simulink model "myo_sfun_one_myo_imu_emg"  (R2019a)
(part 7 of 12)

  "IW{2,1}(59,:)'" : Constant  Value=[0.495840889179216037785380422064918093383312225341796875;1.1802197945522425737152616420644335448741912841796875;0.561954816977624727059037468279711902141571044921875;-1.53262922594306960633048220188356935977935791015625;-1.142041866402901728605456810328178107738494873046875;0.444427633542582134484888456427142955362796783447265625;-1.8064715262999488931683345072087831795215606689453125;1.404352830198885460077917741728015244007110595703125]
      mask Display: e = 0.06;c1 = [120 150 230]/255;c2 = ([120 150 230]+0)/383;c3 = ([120 150 230]+128)/383;patch([0 1 1 0],[0 0 1 1],c1);patch([0 1 1 1-e 1-e 0+e],[0 0 1 1-e 0+e 0+e],c2);patch([0 0 1 1-e 0+e 0+e],[0 1 1 1-e 1-e 0+e],c3);plot([0 1 1 0 0],[0 0 1 1 0]);disp('weights');
  "IW{2,1}(590,:)'" : Constant  Value=[1.1365588902599637055601533575099892914295196533203125;-0.7779843835963247133946651956648565828800201416015625;-1.61735271565704774587857173173688352108001708984375;-1.546406279871038957907103394973091781139373779296875;-1.3702407717835847211773625531350262463092803955078125;-0.83551628178603365437737693355302326381206512451171875;0.34674347307820341246298312398721463978290557861328125;1.31964609753725081731090540415607392787933349609375]
      mask Display: e = 0.06;c1 = [120 150 230]/255;c2 = ([120 150 230]+0)/383;c3 = ([120 150 230]+128)/383;patch([0 1 1 0],[0 0 1 1],c1);patch([0 1 1 1-e 1-e 0+e],[0 0 1 1-e 0+e 0+e],c2);patch([0 0 1 1-e 0+e 0+e],[0 1 1 1-e 1-e 0+e],c3);plot([0 1 1 0 0],[0 0 1 1 0]);disp('weights');
  "IW{2,1}(591,:)'" : Constant  Value=[-0.5970468213357691400489102306892164051532745361328125;-0.5252295626150751406413519362104125320911407470703125;0.7731235904409377024393279498326592147350311279296875;1.10843773794026301260373656987212598323822021484375;2.116586324738635394027141956030391156673431396484375;-0.56051950742911482716834825623664073646068572998046875;0.0989810494305454202645933037274517118930816650390625;1.9395521357138549856102827106951735913753509521484375]
      mask Display: e = 0.06;c1 = [120 150 230]/255;c2 = ([120 150 230]+0)/383;c3 = ([120 150 230]+128)/383;patch([0 1 1 0],[0 0 1 1],c1);patch([0 1 1 1-e 1-e 0+e],[0 0 1 1-e 0+e 0+e],c2);patch([0 0 1 1-e 0+e 0+e],[0 1 1 1-e 1-e 0+e],c3);plot([0 1 1 0 0],[0 0 1 1 0]);disp('weights');
  "IW{2,1}(592,:)'" : Constant  Value=[0.56541018625955263843252396327443420886993408203125;-1.92923127145409711857837464776821434497833251953125;-0.11742767155972898274196580814532353542745113372802734375;0.91189640930210702496339081335463561117649078369140625;0.69079553727149856090505863903672434389591217041015625;-1.65512578383373831769631578936241567134857177734375;-1.67777522610076790243738287244923412799835205078125;-0.045770072495004303358978603455398115329444408416748046875]
      mask Display: e = 0.06;c1 = [120 150 230]/255;c2 = ([120 150 230]+0)/383;c3 = ([120 150 230]+128)/383;patch([0 1 1 0],[0 0 1 1],c1);patch([0 1 1 1-e 1-e 0+e],[0 0 1 1-e 0+e 0+e],c2);patch([0 0 1 1-e 0+e 0+e],[0 1 1 1-e 1-e 0+e],c3);plot([0 1 1 0 0],[0 0 1 1 0]);disp('weights');
  "IW{2,1}(593,:)'" : Constant  Value=[1.631995878217446627189701757743023335933685302734375;0.354312519105268231012217938769026659429073333740234375;-0.110400014047913275216927786459564231336116790771484375;1.975595419315174350316510754055343568325042724609375;-0.53976251419960596944491726389969699084758758544921875;-1.4102684742488220681622124175191856920719146728515625;-0.967888206577956378140470405924133956432342529296875;1.0042302158486886565214035726967267692089080810546875]
      mask Display: e = 0.06;c1 = [120 150 230]/255;c2 = ([120 150 230]+0)/383;c3 = ([120 150 230]+128)/383;patch([0 1 1 0],[0 0 1 1],c1);patch([0 1 1 1-e 1-e 0+e],[0 0 1 1-e 0+e 0+e],c2);patch([0 0 1 1-e 0+e 0+e],[0 1 1 1-e 1-e 0+e],c3);plot([0 1 1 0 0],[0 0 1 1 0]);disp('weights');
  "IW{2,1}(594,:)'" : Constant  Value=[1.362855066833854156271854662918485701084136962890625;-1.01753460758354652426760367234237492084503173828125;0.29473268723076551101058839776669628918170928955078125;-0.60966157783774022060896413677255623042583465576171875;-1.3137337831112760877516620894311927258968353271484375;1.764809052114024279234172354335896670818328857421875;1.3718061592596015874079284913023002445697784423828125;0.97264122462135294000518115353770554065704345703125]
      mask Display: e = 0.06;c1 = [120 150 230]/255;c2 = ([120 150 230]+0)/383;c3 = ([120 150 230]+128)/383;patch([0 1 1 0],[0 0 1 1],c1);patch([0 1 1 1-e 1-e 0+e],[0 0 1 1-e 0+e 0+e],c2);patch([0 0 1 1-e 0+e 0+e],[0 1 1 1-e 1-e 0+e],c3);plot([0 1 1 0 0],[0 0 1 1 0]);disp('weights');
  "IW{2,1}(595,:)'" : Constant  Value=[1.7846936263903485642146051759482361376285552978515625;1.17349851398560556248185093863867223262786865234375;1.23537906283144938157647629850544035434722900390625;0.3825987556562269187310221241204999387264251708984375;-1.2332173382475872802643834802438504993915557861328125;0.11657394714668019297665324529589270241558551788330078125;1.813627133167102556399186141788959503173828125;0.0224668411552899037475494736781911342404782772064208984375]
      mask Display: e = 0.06;c1 = [120 150 230]/255;c2 = ([120 150 230]+0)/383;c3 = ([120 150 230]+128)/383;patch([0 1 1 0],[0 0 1 1],c1);patch([0 1 1 1-e 1-e 0+e],[0 0 1 1-e 0+e 0+e],c2);patch([0 0 1 1-e 0+e 0+e],[0 1 1 1-e 1-e 0+e],c3);plot([0 1 1 0 0],[0 0 1 1 0]);disp('weights');
  "IW{2,1}(596,:)'" : Constant  Value=[-2.033022840198186020899129289318807423114776611328125;1.079443546648902074736042777658440172672271728515625;-0.1575933052745503160085860372419119812548160552978515625;-0.547083934928751514092937213717959821224212646484375;1.4229208556832853016516082789166830480098724365234375;-1.5372500566353324291668513978947885334491729736328125;-0.94194300770826944191327356747933663427829742431640625;-0.33000270358517547197862995744799263775348663330078125]
      mask Display: e = 0.06;c1 = [120 150 230]/255;c2 = ([120 150 230]+0)/383;c3 = ([120 150 230]+128)/383;patch([0 1 1 0],[0 0 1 1],c1);patch([0 1 1 1-e 1-e 0+e],[0 0 1 1-e 0+e 0+e],c2);patch([0 0 1 1-e 0+e 0+e],[0 1 1 1-e 1-e 0+e],c3);plot([0 1 1 0 0],[0 0 1 1 0]);disp('weights');
  "IW{2,1}(597,:)'" : Constant  Value=[2.77675076351304550570375795359723269939422607421875;-0.1567492229542953585674780470071709714829921722412109375;0.76572830357359944475348356718313880264759063720703125;-0.13117528257276733771874432932236231863498687744140625;1.034684891448059307350604285602457821369171142578125;0.210211678674975088743082096698344685137271881103515625;-0.987697962369239679247812091489322483539581298828125;0.741366082034913720377744539291597902774810791015625]
      mask Display: e = 0.06;c1 = [120 150 230]/255;c2 = ([120 150 230]+0)/383;c3 = ([120 150 230]+128)/383;patch([0 1 1 0],[0 0 1 1],c1);patch([0 1 1 1-e 1-e 0+e],[0 0 1 1-e 0+e 0+e],c2);patch([0 0 1 1-e 0+e 0+e],[0 1 1 1-e 1-e 0+e],c3);plot([0 1 1 0 0],[0 0 1 1 0]);disp('weights');
  "IW{2,1}(598,:)'" : Constant  Value=[-1.4404722918007439869114705288666300475597381591796875;1.4952177887590389904204357662820257246494293212890625;0.7882227735106985822000069674686528742313385009765625;1.250002842826308135926183240371756255626678466796875;-0.240822773039876258938107866924838162958621978759765625;-1.3647491667626006073277267205412499606609344482421875;-1.4597226525156685728035199645091779530048370361328125;0.7848545039343071128001838587806560099124908447265625]
      mask Display: e = 0.06;c1 = [120 150 230]/255;c2 = ([120 150 230]+0)/383;c3 = ([120 150 230]+128)/383;patch([0 1 1 0],[0 0 1 1],c1);patch([0 1 1 1-e 1-e 0+e],[0 0 1 1-e 0+e 0+e],c2);patch([0 0 1 1-e 0+e 0+e],[0 1 1 1-e 1-e 0+e],c3);plot([0 1 1 0 0],[0 0 1 1 0]);disp('weights');
  "IW{2,1}(599,:)'" : Constant  Value=[1.3324967037313222295580317222629673779010772705078125;1.9427219282712944181668035525945015251636505126953125;-0.246444365406416066033301603965810500085353851318359375;1.03972745733009386270850882283411920070648193359375;0.94374530422070801449763166601769626140594482421875;-1.5873018147496045227029526358819566667079925537109375;0.4525167778451917310889029977261088788509368896484375;-0.8947395514296709873036661520018242299556732177734375]
      mask Display: e = 0.06;c1 = [120 150 230]/255;c2 = ([120 150 230]+0)/383;c3 = ([120 150 230]+128)/383;patch([0 1 1 0],[0 0 1 1],c1);patch([0 1 1 1-e 1-e 0+e],[0 0 1 1-e 0+e 0+e],c2);patch([0 0 1 1-e 0+e 0+e],[0 1 1 1-e 1-e 0+e],c3);plot([0 1 1 0 0],[0 0 1 1 0]);disp('weights');
  "IW{2,1}(6,:)'" : Constant  Value=[1.3989645708381897026839624231797643005847930908203125;0.878871965177622005427338081062771379947662353515625;1.4478398212565826153053194502717815339565277099609375;0.386861724085491631708322302074520848691463470458984375;-1.4881625315723978619786294075311161577701568603515625;1.25220042774751139091904406086541712284088134765625;-1.41799544675611599586773081682622432708740234375;-0.450735541140858231301535852253437042236328125]
      mask Display: e = 0.06;c1 = [120 150 230]/255;c2 = ([120 150 230]+0)/383;c3 = ([120 150 230]+128)/383;patch([0 1 1 0],[0 0 1 1],c1);patch([0 1 1 1-e 1-e 0+e],[0 0 1 1-e 0+e 0+e],c2);patch([0 0 1 1-e 0+e 0+e],[0 1 1 1-e 1-e 0+e],c3);plot([0 1 1 0 0],[0 0 1 1 0]);disp('weights');
  "IW{2,1}(60,:)'" : Constant  Value=[-1.56723963251996156742507082526572048664093017578125;-1.8273391712930813213233705027960240840911865234375;0.062222286282019624581440808697152533568441867828369140625;0.489904984279520616663461396456114016473293304443359375;0.263246879203439199113034874244476668536663055419921875;-1.783690226821929680767198078683577477931976318359375;-0.3950211766085482967270081644528545439243316650390625;-1.305120998374337037972736652591265738010406494140625]
      mask Display: e = 0.06;c1 = [120 150 230]/255;c2 = ([120 150 230]+0)/383;c3 = ([120 150 230]+128)/383;patch([0 1 1 0],[0 0 1 1],c1);patch([0 1 1 1-e 1-e 0+e],[0 0 1 1-e 0+e 0+e],c2);patch([0 0 1 1-e 0+e 0+e],[0 1 1 1-e 1-e 0+e],c3);plot([0 1 1 0 0],[0 0 1 1 0]);disp('weights');
  "IW{2,1}(600,:)'" : Constant  Value=[0.1399013578316503358944800083918380551040172576904296875;0.994745433658990041436709361732937395572662353515625;0.07987948964757167480410515736366505734622478485107421875;-1.1014921740343570633058334351517260074615478515625;0.90693688484948487005254946780041791498661041259765625;-2.023313920340508165196524714701808989048004150390625;0.2991665154529716819098439373192377388477325439453125;1.9577441671871154138528936528018675744533538818359375]
      mask Display: e = 0.06;c1 = [120 150 230]/255;c2 = ([120 150 230]+0)/383;c3 = ([120 150 230]+128)/383;patch([0 1 1 0],[0 0 1 1],c1);patch([0 1 1 1-e 1-e 0+e],[0 0 1 1-e 0+e 0+e],c2);patch([0 0 1 1-e 0+e 0+e],[0 1 1 1-e 1-e 0+e],c3);plot([0 1 1 0 0],[0 0 1 1 0]);disp('weights');
  "IW{2,1}(601,:)'" : Constant  Value=[-1.0462262509493889250933307266677729785442352294921875;-1.363451040177134476749642999493516981601715087890625;-1.3802141630787783110889677118393592536449432373046875;-1.4657412561269500539395949090248905122280120849609375;1.27038054359856733555034224991686642169952392578125;-0.59673781341977327752346127454075030982494354248046875;1.4209709404646198027677428399329073727130889892578125;0.186387720666462197716128912361455149948596954345703125]
      mask Display: e = 0.06;c1 = [120 150 230]/255;c2 = ([120 150 230]+0)/383;c3 = ([120 150 230]+128)/383;patch([0 1 1 0],[0 0 1 1],c1);patch([0 1 1 1-e 1-e 0+e],[0 0 1 1-e 0+e 0+e],c2);patch([0 0 1 1-e 0+e 0+e],[0 1 1 1-e 1-e 0+e],c3);plot([0 1 1 0 0],[0 0 1 1 0]);disp('weights');
  "IW{2,1}(602,:)'" : Constant  Value=[1.0676591676437723332782070428947918117046356201171875;-1.1515456246222381953003832677495665848255157470703125;1.199234109027186523377395133138634264469146728515625;1.1004753429431255451476090456708334386348724365234375;0.348101446973952344254854551763855852186679840087890625;1.257095724948527060149672252009622752666473388671875;1.536305124972318747467170396703295409679412841796875;1.3476924591500065719884560166974551975727081298828125]
      mask Display: e = 0.06;c1 = [120 150 230]/255;c2 = ([120 150 230]+0)/383;c3 = ([120 150 230]+128)/383;patch([0 1 1 0],[0 0 1 1],c1);patch([0 1 1 1-e 1-e 0+e],[0 0 1 1-e 0+e 0+e],c2);patch([0 0 1 1-e 0+e 0+e],[0 1 1 1-e 1-e 0+e],c3);plot([0 1 1 0 0],[0 0 1 1 0]);disp('weights');
  "IW{2,1}(603,:)'" : Constant  Value=[-0.8102015609143695673566298864898271858692169189453125;0.9788842783427773586168996189371682703495025634765625;-0.546574779209751948627626916277222335338592529296875;-1.380296283345530117259158942033536732196807861328125;-1.3637937080773421261170597063028253614902496337890625;1.5946411678625553864918629187741316854953765869140625;0.94363969580705742146164993755519390106201171875;-1.43620112704588986929366001277230679988861083984375]
      mask Display: e = 0.06;c1 = [120 150 230]/255;c2 = ([120 150 230]+0)/383;c3 = ([120 150 230]+128)/383;patch([0 1 1 0],[0 0 1 1],c1);patch([0 1 1 1-e 1-e 0+e],[0 0 1 1-e 0+e 0+e],c2);patch([0 0 1 1-e 0+e 0+e],[0 1 1 1-e 1-e 0+e],c3);plot([0 1 1 0 0],[0 0 1 1 0]);disp('weights');
  "IW{2,1}(604,:)'" : Constant  Value=[0.406274079118545572431031587257166393101215362548828125;-1.0380674950344452867057043476961553096771240234375;1.3401458758174744634317221425590105354785919189453125;-0.44440858715460251904261212985147722065448760986328125;0.97805948319445568106544897091225720942020416259765625;-1.065572892148696215741665582754649221897125244140625;1.7562937018632605035151073025190271437168121337890625;-1.6116834669183486283827733132056891918182373046875]
      mask Display: e = 0.06;c1 = [120 150 230]/255;c2 = ([120 150 230]+0)/383;c3 = ([120 150 230]+128)/383;patch([0 1 1 0],[0 0 1 1],c1);patch([0 1 1 1-e 1-e 0+e],[0 0 1 1-e 0+e 0+e],c2);patch([0 0 1 1-e 0+e 0+e],[0 1 1 1-e 1-e 0+e],c3);plot([0 1 1 0 0],[0 0 1 1 0]);disp('weights');
  "IW{2,1}(605,:)'" : Constant  Value=[0.744501259166927109589551037061028182506561279296875;-1.160653386032304279495974697056226432323455810546875;1.663776115535684052559872725396417081356048583984375;0.08145048492487029501152306920630508102476596832275390625;1.5551761046942977895213289230014197528362274169921875;1.6110581647783417391650573335937224328517913818359375;-0.77332975038642615128736679253051988780498504638671875;-0.86635308081110107281119780964218080043792724609375]
      mask Display: e = 0.06;c1 = [120 150 230]/255;c2 = ([120 150 230]+0)/383;c3 = ([120 150 230]+128)/383;patch([0 1 1 0],[0 0 1 1],c1);patch([0 1 1 1-e 1-e 0+e],[0 0 1 1-e 0+e 0+e],c2);patch([0 0 1 1-e 0+e 0+e],[0 1 1 1-e 1-e 0+e],c3);plot([0 1 1 0 0],[0 0 1 1 0]);disp('weights');
  "IW{2,1}(606,:)'" : Constant  Value=[-2.00759017283681817644946931977756321430206298828125;1.4790292348892355445144630721188150346279144287109375;0.9381068897441531273528880774392746388912200927734375;-1.0279233837163934683900379241094924509525299072265625;1.530338655101361577948182457475923001766204833984375;0.70558561888594562017118505536927841603755950927734375;-0.389949820912730060751272276320378296077251434326171875;-0.30903615573059750598616801653406582772731781005859375]
      mask Display: e = 0.06;c1 = [120 150 230]/255;c2 = ([120 150 230]+0)/383;c3 = ([120 150 230]+128)/383;patch([0 1 1 0],[0 0 1 1],c1);patch([0 1 1 1-e 1-e 0+e],[0 0 1 1-e 0+e 0+e],c2);patch([0 0 1 1-e 0+e 0+e],[0 1 1 1-e 1-e 0+e],c3);plot([0 1 1 0 0],[0 0 1 1 0]);disp('weights');
  "IW{2,1}(607,:)'" : Constant  Value=[-1.0176822149305377873673705835244618356227874755859375;-0.88067083235813570230021696261246688663959503173828125;-1.2233134249827359862905495901941321790218353271484375;1.6120984193939709161469409082201309502124786376953125;-0.01641788180701951593842835563918924890458583831787109375;1.842094851055680493345789727754890918731689453125;0.387559764525972905158113235302153043448925018310546875;-1.28754911299864627238775938167236745357513427734375]
      mask Display: e = 0.06;c1 = [120 150 230]/255;c2 = ([120 150 230]+0)/383;c3 = ([120 150 230]+128)/383;patch([0 1 1 0],[0 0 1 1],c1);patch([0 1 1 1-e 1-e 0+e],[0 0 1 1-e 0+e 0+e],c2);patch([0 0 1 1-e 0+e 0+e],[0 1 1 1-e 1-e 0+e],c3);plot([0 1 1 0 0],[0 0 1 1 0]);disp('weights');
  "IW{2,1}(608,:)'" : Constant  Value=[0.06756783426557622096453314952668733894824981689453125;-0.97985811135812161953850818463251926004886627197265625;1.9165656766479255423973881988786160945892333984375;0.97999553847674636397613312510657124221324920654296875;1.0965168003811542885017615844844840466976165771484375;0.91483034898736093065707564164767973124980926513671875;0.416384344635610970097872041151276789605617523193359375;-1.8438560716209162482215333511703647673130035400390625]
      mask Display: e = 0.06;c1 = [120 150 230]/255;c2 = ([120 150 230]+0)/383;c3 = ([120 150 230]+128)/383;patch([0 1 1 0],[0 0 1 1],c1);patch([0 1 1 1-e 1-e 0+e],[0 0 1 1-e 0+e 0+e],c2);patch([0 0 1 1-e 0+e 0+e],[0 1 1 1-e 1-e 0+e],c3);plot([0 1 1 0 0],[0 0 1 1 0]);disp('weights');
  "IW{2,1}(609,:)'" : Constant  Value=[0.90824883915620002738933180808089673519134521484375;1.5432188808015123715478011945378966629505157470703125;-0.484591429101132231682669271322083659470081329345703125;-0.75644137307587389074114980758167803287506103515625;-1.4204857677377356051096057854010723531246185302734375;1.5424089274776846547609920889954082667827606201171875;-1.3677706917546246234707041367073543369770050048828125;0.67875477880856471823989295444334857165813446044921875]
      mask Display: e = 0.06;c1 = [120 150 230]/255;c2 = ([120 150 230]+0)/383;c3 = ([120 150 230]+128)/383;patch([0 1 1 0],[0 0 1 1],c1);patch([0 1 1 1-e 1-e 0+e],[0 0 1 1-e 0+e 0+e],c2);patch([0 0 1 1-e 0+e 0+e],[0 1 1 1-e 1-e 0+e],c3);plot([0 1 1 0 0],[0 0 1 1 0]);disp('weights');
  "IW{2,1}(61,:)'" : Constant  Value=[-0.583346229666195537078010602272115647792816162109375;0.652606918201581009952860767953097820281982421875;1.54396791785674469821287857485003769397735595703125;-0.8547845495893435785461633713566698133945465087890625;1.440314162861167091023162356577813625335693359375;0.48672290195644507537764411608804948627948760986328125;-1.430158866254590321887008030898869037628173828125;1.66829878736194192612174447276629507541656494140625]
      mask Display: e = 0.06;c1 = [120 150 230]/255;c2 = ([120 150 230]+0)/383;c3 = ([120 150 230]+128)/383;patch([0 1 1 0],[0 0 1 1],c1);patch([0 1 1 1-e 1-e 0+e],[0 0 1 1-e 0+e 0+e],c2);patch([0 0 1 1-e 0+e 0+e],[0 1 1 1-e 1-e 0+e],c3);plot([0 1 1 0 0],[0 0 1 1 0]);disp('weights');
  "IW{2,1}(610,:)'" : Constant  Value=[1.0695065922145297054868251507286913692951202392578125;-0.5602414711219931842123287424328736960887908935546875;1.564508360252296004233585335896350443363189697265625;0.443578046982452567359445083639002405107021331787109375;1.8320578553493607198987547235446982085704803466796875;0.2373867145462984218351465415253187529742717742919921875;-1.4201256732646430069877396817901171743869781494140625;-1.230718785601741416257937089540064334869384765625]
      mask Display: e = 0.06;c1 = [120 150 230]/255;c2 = ([120 150 230]+0)/383;c3 = ([120 150 230]+128)/383;patch([0 1 1 0],[0 0 1 1],c1);patch([0 1 1 1-e 1-e 0+e],[0 0 1 1-e 0+e 0+e],c2);patch([0 0 1 1-e 0+e 0+e],[0 1 1 1-e 1-e 0+e],c3);plot([0 1 1 0 0],[0 0 1 1 0]);disp('weights');
  "IW{2,1}(611,:)'" : Constant  Value=[-0.56186312548356831531037869353895075619220733642578125;1.9518020246530098926740492970566265285015106201171875;-0.94334391080466650780778081752941943705081939697265625;-1.9538154513649264032437713467516005039215087890625;0.109136425671035930395902369127725251019001007080078125;-0.528305999598769115976892862818203866481781005859375;0.8902645159678039821216088967048563063144683837890625;1.022948550793317590290598673163913190364837646484375]
      mask Display: e = 0.06;c1 = [120 150 230]/255;c2 = ([120 150 230]+0)/383;c3 = ([120 150 230]+128)/383;patch([0 1 1 0],[0 0 1 1],c1);patch([0 1 1 1-e 1-e 0+e],[0 0 1 1-e 0+e 0+e],c2);patch([0 0 1 1-e 0+e 0+e],[0 1 1 1-e 1-e 0+e],c3);plot([0 1 1 0 0],[0 0 1 1 0]);disp('weights');
  "IW{2,1}(612,:)'" : Constant  Value=[-1.19478104240437144056841134442947804927825927734375;2.162698980018332495234290036023594439029693603515625;-0.693116982716233120953575053135864436626434326171875;1.2670612929229212451076591605669818818569183349609375;1.154640366877071944173849260550923645496368408203125;-0.618604838251085364930759169510565698146820068359375;0.318475683817145138743143206738750450313091278076171875;-0.99402698682691192910709787611267529428005218505859375]
      mask Display: e = 0.06;c1 = [120 150 230]/255;c2 = ([120 150 230]+0)/383;c3 = ([120 150 230]+128)/383;patch([0 1 1 0],[0 0 1 1],c1);patch([0 1 1 1-e 1-e 0+e],[0 0 1 1-e 0+e 0+e],c2);patch([0 0 1 1-e 0+e 0+e],[0 1 1 1-e 1-e 0+e],c3);plot([0 1 1 0 0],[0 0 1 1 0]);disp('weights');
  "IW{2,1}(613,:)'" : Constant  Value=[1.5390431098582713076439176802523434162139892578125;0.311842151138437662094560209880000911653041839599609375;-0.432826553257930901619232599841780029237270355224609375;-1.135667286790710051036512595601379871368408203125;-1.2510952563992765451672539711580611765384674072265625;-1.099051054945733074674762974609620869159698486328125;-1.314184632408988750995604277704842388629913330078125;-1.5719194667600806525342704844661056995391845703125]
      mask Display: e = 0.06;c1 = [120 150 230]/255;c2 = ([120 150 230]+0)/383;c3 = ([120 150 230]+128)/383;patch([0 1 1 0],[0 0 1 1],c1);patch([0 1 1 1-e 1-e 0+e],[0 0 1 1-e 0+e 0+e],c2);patch([0 0 1 1-e 0+e 0+e],[0 1 1 1-e 1-e 0+e],c3);plot([0 1 1 0 0],[0 0 1 1 0]);disp('weights');
  "IW{2,1}(614,:)'" : Constant  Value=[0.415642840330518958946726115755154751241207122802734375;1.47348021001815165931247975095175206661224365234375;0.5290336561264969983398032127297483384609222412109375;-1.3355131601420442422067935694940388202667236328125;1.91821924338969385104292086907662451267242431640625;0.598986782930229555432788401958532631397247314453125;-1.395334022050206623788426441024057567119598388671875;-0.83432116509932086056977595944772474467754364013671875]
      mask Display: e = 0.06;c1 = [120 150 230]/255;c2 = ([120 150 230]+0)/383;c3 = ([120 150 230]+128)/383;patch([0 1 1 0],[0 0 1 1],c1);patch([0 1 1 1-e 1-e 0+e],[0 0 1 1-e 0+e 0+e],c2);patch([0 0 1 1-e 0+e 0+e],[0 1 1 1-e 1-e 0+e],c3);plot([0 1 1 0 0],[0 0 1 1 0]);disp('weights');
  "IW{2,1}(615,:)'" : Constant  Value=[-0.9243394765822106062813645621645264327526092529296875;2.523292336225384957515416317619383335113525390625;-0.497732778806864839538093292503617703914642333984375;1.3000054053377587681694649290875531733036041259765625;0.8499300349543557064890819674474187195301055908203125;0.86402793265875355022131998339318670332431793212890625;-0.57755068516618124352390850617666728794574737548828125;0.1895537067373020134741778974785120226442813873291015625]
      mask Display: e = 0.06;c1 = [120 150 230]/255;c2 = ([120 150 230]+0)/383;c3 = ([120 150 230]+128)/383;patch([0 1 1 0],[0 0 1 1],c1);patch([0 1 1 1-e 1-e 0+e],[0 0 1 1-e 0+e 0+e],c2);patch([0 0 1 1-e 0+e 0+e],[0 1 1 1-e 1-e 0+e],c3);plot([0 1 1 0 0],[0 0 1 1 0]);disp('weights');
  "IW{2,1}(616,:)'" : Constant  Value=[-1.7980650129034174700137782565434463322162628173828125;-0.52787175708551858921424582149484194815158843994140625;0.3999021950203929254286094874260015785694122314453125;1.2856492697510863987275797626352868974208831787109375;-0.8074119078345536326679621197399683296680450439453125;1.0282666253705297076947999812546186149120330810546875;1.5670907494630854639439121456234715878963470458984375;1.2173301229011121993295319043681956827640533447265625]
      mask Display: e = 0.06;c1 = [120 150 230]/255;c2 = ([120 150 230]+0)/383;c3 = ([120 150 230]+128)/383;patch([0 1 1 0],[0 0 1 1],c1);patch([0 1 1 1-e 1-e 0+e],[0 0 1 1-e 0+e 0+e],c2);patch([0 0 1 1-e 0+e 0+e],[0 1 1 1-e 1-e 0+e],c3);plot([0 1 1 0 0],[0 0 1 1 0]);disp('weights');
  "IW{2,1}(617,:)'" : Constant  Value=[0.8233944981282481645479265353060327470302581787109375;2.07864078264244600546817309805192053318023681640625;0.97238679166842933998538001105771400034427642822265625;-0.7199181388481150634106597863137722015380859375;0.421549209390107371131506397432531230151653289794921875;-1.1523597959586282524213629585574381053447723388671875;-0.425262518672025635613209715302218683063983917236328125;-1.6941255159399364327299508659052662551403045654296875]
      mask Display: e = 0.06;c1 = [120 150 230]/255;c2 = ([120 150 230]+0)/383;c3 = ([120 150 230]+128)/383;patch([0 1 1 0],[0 0 1 1],c1);patch([0 1 1 1-e 1-e 0+e],[0 0 1 1-e 0+e 0+e],c2);patch([0 0 1 1-e 0+e 0+e],[0 1 1 1-e 1-e 0+e],c3);plot([0 1 1 0 0],[0 0 1 1 0]);disp('weights');
  "IW{2,1}(618,:)'" : Constant  Value=[-1.3845112013980223064635310947778634727001190185546875;1.2581019145671932246699498136877082288265228271484375;0.385219614654531194997133525248500518500804901123046875;-0.378698122941593329215947960619814693927764892578125;1.6636808845950714630390621096012182533740997314453125;-1.326437238051724865073310866137035191059112548828125;-0.4094163915923871854829485528171062469482421875;1.599983886636860308527730012428946793079376220703125]
      mask Display: e = 0.06;c1 = [120 150 230]/255;c2 = ([120 150 230]+0)/383;c3 = ([120 150 230]+128)/383;patch([0 1 1 0],[0 0 1 1],c1);patch([0 1 1 1-e 1-e 0+e],[0 0 1 1-e 0+e 0+e],c2);patch([0 0 1 1-e 0+e 0+e],[0 1 1 1-e 1-e 0+e],c3);plot([0 1 1 0 0],[0 0 1 1 0]);disp('weights');
  "IW{2,1}(619,:)'" : Constant  Value=[1.6832996710298167020170012619928456842899322509765625;0.449539198982113585856268400675617158412933349609375;0.8307320998601823713869407583842985332012176513671875;-0.6832544444925467974627508738194592297077178955078125;-2.2669423406538786736064139404334127902984619140625;-0.21058789806763034135883572162128984928131103515625;-0.93104019495121892457945023124921135604381561279296875;-0.94874025383826599000514079307322390377521514892578125]
      mask Display: e = 0.06;c1 = [120 150 230]/255;c2 = ([120 150 230]+0)/383;c3 = ([120 150 230]+128)/383;patch([0 1 1 0],[0 0 1 1],c1);patch([0 1 1 1-e 1-e 0+e],[0 0 1 1-e 0+e 0+e],c2);patch([0 0 1 1-e 0+e 0+e],[0 1 1 1-e 1-e 0+e],c3);plot([0 1 1 0 0],[0 0 1 1 0]);disp('weights');
  "IW{2,1}(62,:)'" : Constant  Value=[-0.80784071268572432700239005498588085174560546875;-0.86454159290918097813261056217015720903873443603515625;-1.02798280810631492698803413077257573604583740234375;-0.843159200916097528732962018693797290325164794921875;1.9764345113544423693241469663917087018489837646484375;-1.0226218063283021297849018083070404827594757080078125;1.3440794621918434881280290937866084277629852294921875;-1.0325956562448708186963131083757616579532623291015625]
      mask Display: e = 0.06;c1 = [120 150 230]/255;c2 = ([120 150 230]+0)/383;c3 = ([120 150 230]+128)/383;patch([0 1 1 0],[0 0 1 1],c1);patch([0 1 1 1-e 1-e 0+e],[0 0 1 1-e 0+e 0+e],c2);patch([0 0 1 1-e 0+e 0+e],[0 1 1 1-e 1-e 0+e],c3);plot([0 1 1 0 0],[0 0 1 1 0]);disp('weights');
  "IW{2,1}(620,:)'" : Constant  Value=[1.334947324367666166011758832610212266445159912109375;-1.3273493586359659257567500389995984733104705810546875;-0.1321542017070956587243557578403851948678493499755859375;-1.294590725841910927584876844775862991809844970703125;1.4144908241846343432968069464550353586673736572265625;-0.4990548052459355954368902530404739081859588623046875;-1.14994285385152839040756589383818209171295166015625;-1.4414002009392941072718485884252004325389862060546875]
      mask Display: e = 0.06;c1 = [120 150 230]/255;c2 = ([120 150 230]+0)/383;c3 = ([120 150 230]+128)/383;patch([0 1 1 0],[0 0 1 1],c1);patch([0 1 1 1-e 1-e 0+e],[0 0 1 1-e 0+e 0+e],c2);patch([0 0 1 1-e 0+e 0+e],[0 1 1 1-e 1-e 0+e],c3);plot([0 1 1 0 0],[0 0 1 1 0]);disp('weights');
  "IW{2,1}(621,:)'" : Constant  Value=[-0.1155194033765267469515691800552303902804851531982421875;-0.344314053861413338353258950519375503063201904296875;-0.18025558100015171003605018995585851371288299560546875;1.66092833072870948996069273562170565128326416015625;0.5727993422400086132029173313640058040618896484375;1.389429199332991249349333884310908615589141845703125;0.5034936486076386774612956287455745041370391845703125;-2.326123140285625279233272522105835378170013427734375]
      mask Display: e = 0.06;c1 = [120 150 230]/255;c2 = ([120 150 230]+0)/383;c3 = ([120 150 230]+128)/383;patch([0 1 1 0],[0 0 1 1],c1);patch([0 1 1 1-e 1-e 0+e],[0 0 1 1-e 0+e 0+e],c2);patch([0 0 1 1-e 0+e 0+e],[0 1 1 1-e 1-e 0+e],c3);plot([0 1 1 0 0],[0 0 1 1 0]);disp('weights');
  "IW{2,1}(622,:)'" : Constant  Value=[-0.327523627563958752428874277029535733163356781005859375;-1.3950088720842390710430436229216866195201873779296875;-0.07732020025750445391121701277370448224246501922607421875;-1.1070020699473712699756333677214570343494415283203125;1.3609328905626727479472037884988822042942047119140625;1.5808360841818320796647867609863169491291046142578125;1.00853180773224249122677065315656363964080810546875;1.49164411309901101532204847899265587329864501953125]
      mask Display: e = 0.06;c1 = [120 150 230]/255;c2 = ([120 150 230]+0)/383;c3 = ([120 150 230]+128)/383;patch([0 1 1 0],[0 0 1 1],c1);patch([0 1 1 1-e 1-e 0+e],[0 0 1 1-e 0+e 0+e],c2);patch([0 0 1 1-e 0+e 0+e],[0 1 1 1-e 1-e 0+e],c3);plot([0 1 1 0 0],[0 0 1 1 0]);disp('weights');
  "IW{2,1}(623,:)'" : Constant  Value=[0.50926268929817919417502025680732913315296173095703125;1.02354553421339034002812695689499378204345703125;0.4587054237810974655076279304921627044677734375;-1.2664756748000687291977328641223721206188201904296875;-1.0326915158366702929271241373498924076557159423828125;0.404808695052300715477855419521802105009555816650390625;1.7725295585873281911659660181612707674503326416015625;-1.9056231855257212970400360063649713993072509765625]
      mask Display: e = 0.06;c1 = [120 150 230]/255;c2 = ([120 150 230]+0)/383;c3 = ([120 150 230]+128)/383;patch([0 1 1 0],[0 0 1 1],c1);patch([0 1 1 1-e 1-e 0+e],[0 0 1 1-e 0+e 0+e],c2);patch([0 0 1 1-e 0+e 0+e],[0 1 1 1-e 1-e 0+e],c3);plot([0 1 1 0 0],[0 0 1 1 0]);disp('weights');
  "IW{2,1}(624,:)'" : Constant  Value=[-0.426022704578880306858224003008217550814151763916015625;1.974465496821880439171081889071501791477203369140625;0.34657118674579923123246771865524351596832275390625;0.97614887195124910856947053616750054061412811279296875;-1.4175229737882946157156993649550713598728179931640625;-1.33353469225431897626776844845153391361236572265625;0.51150649856705754370267413833062164485454559326171875;-1.3644009071495613039104455310734920203685760498046875]
      mask Display: e = 0.06;c1 = [120 150 230]/255;c2 = ([120 150 230]+0)/383;c3 = ([120 150 230]+128)/383;patch([0 1 1 0],[0 0 1 1],c1);patch([0 1 1 1-e 1-e 0+e],[0 0 1 1-e 0+e 0+e],c2);patch([0 0 1 1-e 0+e 0+e],[0 1 1 1-e 1-e 0+e],c3);plot([0 1 1 0 0],[0 0 1 1 0]);disp('weights');
  "IW{2,1}(625,:)'" : Constant  Value=[1.0892807111617666127045822577201761305332183837890625;1.962879653505605670460454348358325660228729248046875;-0.4366435090927993645237847886164672672748565673828125;-1.499077208754342915852930673281662166118621826171875;-1.062067905261328437660495183081366121768951416015625;0.64284583767381631158599475384107790887355804443359375;1.320911793095183472956932746456004679203033447265625;-0.540715402800169275820962866418994963169097900390625]
      mask Display: e = 0.06;c1 = [120 150 230]/255;c2 = ([120 150 230]+0)/383;c3 = ([120 150 230]+128)/383;patch([0 1 1 0],[0 0 1 1],c1);patch([0 1 1 1-e 1-e 0+e],[0 0 1 1-e 0+e 0+e],c2);patch([0 0 1 1-e 0+e 0+e],[0 1 1 1-e 1-e 0+e],c3);plot([0 1 1 0 0],[0 0 1 1 0]);disp('weights');
  "IW{2,1}(626,:)'" : Constant  Value=[-0.0934478463088293798133321388377225957810878753662109375;0.364146124661070602623880176906823180615901947021484375;1.54354569628061089048287612968124449253082275390625;1.1389569591664339132108807461918331682682037353515625;1.551203771758578486839041943312622606754302978515625;-1.5252177846193613053316084915422834455966949462890625;1.4405943699840950689150531616178341209888458251953125;0.70619852150084183595168951796949841082096099853515625]
      mask Display: e = 0.06;c1 = [120 150 230]/255;c2 = ([120 150 230]+0)/383;c3 = ([120 150 230]+128)/383;patch([0 1 1 0],[0 0 1 1],c1);patch([0 1 1 1-e 1-e 0+e],[0 0 1 1-e 0+e 0+e],c2);patch([0 0 1 1-e 0+e 0+e],[0 1 1 1-e 1-e 0+e],c3);plot([0 1 1 0 0],[0 0 1 1 0]);disp('weights');
  "IW{2,1}(627,:)'" : Constant  Value=[0.09219685402307654931153280131184146739542484283447265625;0.07017065301976861679822405903905746527016162872314453125;1.52843238753498145143794317846186459064483642578125;0.965812028758090246327583372476510703563690185546875;2.112261949203092736837561460561119019985198974609375;0.07524462289875240295078384633598034270107746124267578125;1.751589707715766497386766786803491413593292236328125;0.43357744552148413941239368796232156455516815185546875]
      mask Display: e = 0.06;c1 = [120 150 230]/255;c2 = ([120 150 230]+0)/383;c3 = ([120 150 230]+128)/383;patch([0 1 1 0],[0 0 1 1],c1);patch([0 1 1 1-e 1-e 0+e],[0 0 1 1-e 0+e 0+e],c2);patch([0 0 1 1-e 0+e 0+e],[0 1 1 1-e 1-e 0+e],c3);plot([0 1 1 0 0],[0 0 1 1 0]);disp('weights');
  "IW{2,1}(628,:)'" : Constant  Value=[1.6577552297238258294242996271350421011447906494140625;0.51268986432709573453081475236103869974613189697265625;-1.4036568104439470783262322584050707519054412841796875;0.9921396182445401112914851182722486555576324462890625;-1.53525969285640417894001075183041393756866455078125;1.2058938538982564292467714039958082139492034912109375;0.051529486221002528123502628432106575928628444671630859375;1.091902940613427741567420525825582444667816162109375]
      mask Display: e = 0.06;c1 = [120 150 230]/255;c2 = ([120 150 230]+0)/383;c3 = ([120 150 230]+128)/383;patch([0 1 1 0],[0 0 1 1],c1);patch([0 1 1 1-e 1-e 0+e],[0 0 1 1-e 0+e 0+e],c2);patch([0 0 1 1-e 0+e 0+e],[0 1 1 1-e 1-e 0+e],c3);plot([0 1 1 0 0],[0 0 1 1 0]);disp('weights');
  "IW{2,1}(629,:)'" : Constant  Value=[1.2589993845590898846609206884750165045261383056640625;1.4979357158170494290772012391244061291217803955078125;-0.90621099390727610778384359946358017623424530029296875;0.97946455928432885063017465654411353170871734619140625;-1.0229675550841654807499025992001406848430633544921875;-1.548306923334317186657926868065260350704193115234375;1.281460062898937213304861870710738003253936767578125;-0.58596677840527833236450305776088498532772064208984375]
      mask Display: e = 0.06;c1 = [120 150 230]/255;c2 = ([120 150 230]+0)/383;c3 = ([120 150 230]+128)/383;patch([0 1 1 0],[0 0 1 1],c1);patch([0 1 1 1-e 1-e 0+e],[0 0 1 1-e 0+e 0+e],c2);patch([0 0 1 1-e 0+e 0+e],[0 1 1 1-e 1-e 0+e],c3);plot([0 1 1 0 0],[0 0 1 1 0]);disp('weights');
  "IW{2,1}(63,:)'" : Constant  Value=[-0.7144457458977411246081601348123513162136077880859375;-0.007298700002133218060762498424764999072067439556121826171875;1.44780006772763325528785571805201470851898193359375;-1.788137173619348541109275174676440656185150146484375;-1.58123753756977425410923387971706688404083251953125;1.55199278995771106082202095421962440013885498046875;-0.5036095123205377444008945531095378100872039794921875;0.09057178325152830111743895713516394607722759246826171875]
      mask Display: e = 0.06;c1 = [120 150 230]/255;c2 = ([120 150 230]+0)/383;c3 = ([120 150 230]+128)/383;patch([0 1 1 0],[0 0 1 1],c1);patch([0 1 1 1-e 1-e 0+e],[0 0 1 1-e 0+e 0+e],c2);patch([0 0 1 1-e 0+e 0+e],[0 1 1 1-e 1-e 0+e],c3);plot([0 1 1 0 0],[0 0 1 1 0]);disp('weights');
  "IW{2,1}(630,:)'" : Constant  Value=[0.0982183466709679320327808227375498972833156585693359375;-0.1268629177400806273823263836675323545932769775390625;-0.300995077456217341449473678949289023876190185546875;2.173761256513340622831265136483125388622283935546875;-1.5145394274333738859894538109074346721172332763671875;1.60123112841297920994065862032584846019744873046875;-0.140390045149285602743560730232275091111660003662109375;1.1047487791690600023031265664030797779560089111328125]
      mask Display: e = 0.06;c1 = [120 150 230]/255;c2 = ([120 150 230]+0)/383;c3 = ([120 150 230]+128)/383;patch([0 1 1 0],[0 0 1 1],c1);patch([0 1 1 1-e 1-e 0+e],[0 0 1 1-e 0+e 0+e],c2);patch([0 0 1 1-e 0+e 0+e],[0 1 1 1-e 1-e 0+e],c3);plot([0 1 1 0 0],[0 0 1 1 0]);disp('weights');
  "IW{2,1}(631,:)'" : Constant  Value=[1.3164862241914558893540743156336247920989990234375;-0.468865499463230361865129225407144986093044281005859375;-1.12740594557454887336689353105612099170684814453125;0.61935334953164922211499288096092641353607177734375;-1.809596865877384885834544547833502292633056640625;-0.86133225167429461333057361116516403853893280029296875;-0.50304123527349775546468890752294100821018218994140625;-1.7703580003685785992928458654205314815044403076171875]
      mask Display: e = 0.06;c1 = [120 150 230]/255;c2 = ([120 150 230]+0)/383;c3 = ([120 150 230]+128)/383;patch([0 1 1 0],[0 0 1 1],c1);patch([0 1 1 1-e 1-e 0+e],[0 0 1 1-e 0+e 0+e],c2);patch([0 0 1 1-e 0+e 0+e],[0 1 1 1-e 1-e 0+e],c3);plot([0 1 1 0 0],[0 0 1 1 0]);disp('weights');
  "IW{2,1}(632,:)'" : Constant  Value=[-1.7529823083935516248033081865287385880947113037109375;-0.05735630449086694115923279468916007317602634429931640625;1.6356853806522633210107642298680730164051055908203125;-1.2340016930803094918900342236156575381755828857421875;0.349419931382872472891421011809143237769603729248046875;-1.7927245380449587930371535549056716263294219970703125;-0.384054188232957061099881457266747020184993743896484375;-0.402560198126120261097327102106646634638309478759765625]
      mask Display: e = 0.06;c1 = [120 150 230]/255;c2 = ([120 150 230]+0)/383;c3 = ([120 150 230]+128)/383;patch([0 1 1 0],[0 0 1 1],c1);patch([0 1 1 1-e 1-e 0+e],[0 0 1 1-e 0+e 0+e],c2);patch([0 0 1 1-e 0+e 0+e],[0 1 1 1-e 1-e 0+e],c3);plot([0 1 1 0 0],[0 0 1 1 0]);disp('weights');
  "IW{2,1}(633,:)'" : Constant  Value=[-0.6545074957008936156199752076645381748676300048828125;1.581480496200238672344084989163093268871307373046875;1.516216943401426764381767497980035841464996337890625;-1.1809908709088359213268404346308670938014984130859375;-0.330350011200674253952769277020706795156002044677734375;-0.88508358035018874776511665913858450949192047119140625;1.2832108773659598455196828581392765045166015625;-1.33441950771778383710852722288109362125396728515625]
      mask Display: e = 0.06;c1 = [120 150 230]/255;c2 = ([120 150 230]+0)/383;c3 = ([120 150 230]+128)/383;patch([0 1 1 0],[0 0 1 1],c1);patch([0 1 1 1-e 1-e 0+e],[0 0 1 1-e 0+e 0+e],c2);patch([0 0 1 1-e 0+e 0+e],[0 1 1 1-e 1-e 0+e],c3);plot([0 1 1 0 0],[0 0 1 1 0]);disp('weights');
  "IW{2,1}(634,:)'" : Constant  Value=[-1.1096216500989715125768952930229716002941131591796875;1.509353123664001206094553708680905401706695556640625;0.2116355737257553937258336418381077237427234649658203125;1.64679265651261186320652996073476970195770263671875;-0.96599040664166901937193188132368959486484527587890625;-0.85577737989780755523128163986257277429103851318359375;1.61504603765871035392365229199640452861785888671875;-0.7301337346279890283540225937031209468841552734375]
      mask Display: e = 0.06;c1 = [120 150 230]/255;c2 = ([120 150 230]+0)/383;c3 = ([120 150 230]+128)/383;patch([0 1 1 0],[0 0 1 1],c1);patch([0 1 1 1-e 1-e 0+e],[0 0 1 1-e 0+e 0+e],c2);patch([0 0 1 1-e 0+e 0+e],[0 1 1 1-e 1-e 0+e],c3);plot([0 1 1 0 0],[0 0 1 1 0]);disp('weights');
  "IW{2,1}(635,:)'" : Constant  Value=[1.6737178380947117517507649608887732028961181640625;0.493128149841237928274750856871833093464374542236328125;0.30292831676543852115202071217936463654041290283203125;-0.1312341269964535650505155217615538276731967926025390625;2.14268527738893599376979182125069200992584228515625;1.1550063802665053724894050901639275252819061279296875;0.73286830646691181190277575296931900084018707275390625;1.1922436553784498958208359908894635736942291259765625]
      mask Display: e = 0.06;c1 = [120 150 230]/255;c2 = ([120 150 230]+0)/383;c3 = ([120 150 230]+128)/383;patch([0 1 1 0],[0 0 1 1],c1);patch([0 1 1 1-e 1-e 0+e],[0 0 1 1-e 0+e 0+e],c2);patch([0 0 1 1-e 0+e 0+e],[0 1 1 1-e 1-e 0+e],c3);plot([0 1 1 0 0],[0 0 1 1 0]);disp('weights');
  "IW{2,1}(636,:)'" : Constant  Value=[0.442570136367288979872824938865960575640201568603515625;-0.98216743051010568787972943027853034436702728271484375;-2.076370097602673325809519155882298946380615234375;0.207723083932460139688913614008924923837184906005859375;1.918558194227907076623296234174631536006927490234375;-1.112875532879665119168066667043603956699371337890625;-0.84727086293803088867804262918070890009403228759765625;-0.0490321665702893316751698193911579437553882598876953125]
      mask Display: e = 0.06;c1 = [120 150 230]/255;c2 = ([120 150 230]+0)/383;c3 = ([120 150 230]+128)/383;patch([0 1 1 0],[0 0 1 1],c1);patch([0 1 1 1-e 1-e 0+e],[0 0 1 1-e 0+e 0+e],c2);patch([0 0 1 1-e 0+e 0+e],[0 1 1 1-e 1-e 0+e],c3);plot([0 1 1 0 0],[0 0 1 1 0]);disp('weights');
  "IW{2,1}(637,:)'" : Constant  Value=[1.3986966552773523186914417237858287990093231201171875;1.05986187898607564505937261856161057949066162109375;1.3499273120555803640030489987111650407314300537109375;1.4392274814640872993010134450742043554782867431640625;-0.53957718762312112392720564457704313099384307861328125;-0.04044660310540572345505694329403922893106937408447265625;1.9189093994139956311784089848515577614307403564453125;0.25487430387456677660651394035085104405879974365234375]
      mask Display: e = 0.06;c1 = [120 150 230]/255;c2 = ([120 150 230]+0)/383;c3 = ([120 150 230]+128)/383;patch([0 1 1 0],[0 0 1 1],c1);patch([0 1 1 1-e 1-e 0+e],[0 0 1 1-e 0+e 0+e],c2);patch([0 0 1 1-e 0+e 0+e],[0 1 1 1-e 1-e 0+e],c3);plot([0 1 1 0 0],[0 0 1 1 0]);disp('weights');
  "IW{2,1}(638,:)'" : Constant  Value=[-0.444035083869290969627030563060543499886989593505859375;-1.4892504808588373776956359506584703922271728515625;2.16597097867957710803921145270578563213348388671875;1.31956583710966324218816225766204297542572021484375;-0.36957621024975095824771642583073116838932037353515625;0.031357734113457776115030384289639187045395374298095703125;1.445832975741484727194574588793329894542694091796875;0.75387142477888968716825957017135806381702423095703125]
      mask Display: e = 0.06;c1 = [120 150 230]/255;c2 = ([120 150 230]+0)/383;c3 = ([120 150 230]+128)/383;patch([0 1 1 0],[0 0 1 1],c1);patch([0 1 1 1-e 1-e 0+e],[0 0 1 1-e 0+e 0+e],c2);patch([0 0 1 1-e 0+e 0+e],[0 1 1 1-e 1-e 0+e],c3);plot([0 1 1 0 0],[0 0 1 1 0]);disp('weights');
  "IW{2,1}(639,:)'" : Constant  Value=[-1.533024683823805300875164903118275105953216552734375;-1.8669193144625697566851840747403912246227264404296875;-0.47032166519244811286881713385810144245624542236328125;-0.997914591266086059562212540186010301113128662109375;-1.8168849185548499036713110399432480335235595703125;-0.07296401165905834484970426956351730041205883026123046875;0.54189692295386338027896044877707026898860931396484375;0.60225261795157469801864635883248411118984222412109375]
      mask Display: e = 0.06;c1 = [120 150 230]/255;c2 = ([120 150 230]+0)/383;c3 = ([120 150 230]+128)/383;patch([0 1 1 0],[0 0 1 1],c1);patch([0 1 1 1-e 1-e 0+e],[0 0 1 1-e 0+e 0+e],c2);patch([0 0 1 1-e 0+e 0+e],[0 1 1 1-e 1-e 0+e],c3);plot([0 1 1 0 0],[0 0 1 1 0]);disp('weights');
  "IW{2,1}(64,:)'" : Constant  Value=[0.12336294406974564197287946853975881822407245635986328125;-1.81195390385953647438554980908520519733428955078125;2.09439953183155136429149933974258601665496826171875;-0.493044516884823480484811852875282056629657745361328125;0.77914195501681671185423283532145433127880096435546875;-0.52538815620041534604212074555107392370700836181640625;1.2650929418019754013613464849186129868030548095703125;-0.754199196274558669728094173478893935680389404296875]
      mask Display: e = 0.06;c1 = [120 150 230]/255;c2 = ([120 150 230]+0)/383;c3 = ([120 150 230]+128)/383;patch([0 1 1 0],[0 0 1 1],c1);patch([0 1 1 1-e 1-e 0+e],[0 0 1 1-e 0+e 0+e],c2);patch([0 0 1 1-e 0+e 0+e],[0 1 1 1-e 1-e 0+e],c3);plot([0 1 1 0 0],[0 0 1 1 0]);disp('weights');
  "IW{2,1}(640,:)'" : Constant  Value=[-0.395647130047409645303702063756645657122135162353515625;0.2073450232209671784122662074878462590277194976806640625;-1.7703354965953941313472341789747588336467742919921875;1.583398856688008837778625093051232397556304931640625;1.7550476267779229200272084199241362512111663818359375;0.7289527801825936847990305977873504161834716796875;0.52488657792418702552339482281240634620189666748046875;1.124080103628520621583675165311433374881744384765625]
      mask Display: e = 0.06;c1 = [120 150 230]/255;c2 = ([120 150 230]+0)/383;c3 = ([120 150 230]+128)/383;patch([0 1 1 0],[0 0 1 1],c1);patch([0 1 1 1-e 1-e 0+e],[0 0 1 1-e 0+e 0+e],c2);patch([0 0 1 1-e 0+e 0+e],[0 1 1 1-e 1-e 0+e],c3);plot([0 1 1 0 0],[0 0 1 1 0]);disp('weights');
  "IW{2,1}(641,:)'" : Constant  Value=[-1.0390123455352793246930787063320167362689971923828125;1.61103604130202260336091057979501783847808837890625;-1.227174710786481881541476468555629253387451171875;1.1827535819958487905978472554124891757965087890625;1.0229356228663013528290548492805100977420806884765625;-0.8655361719209258009044560822076164186000823974609375;1.069378679865401249315937093342654407024383544921875;1.21325907259273169103153122705407440662384033203125]
      mask Display: e = 0.06;c1 = [120 150 230]/255;c2 = ([120 150 230]+0)/383;c3 = ([120 150 230]+128)/383;patch([0 1 1 0],[0 0 1 1],c1);patch([0 1 1 1-e 1-e 0+e],[0 0 1 1-e 0+e 0+e],c2);patch([0 0 1 1-e 0+e 0+e],[0 1 1 1-e 1-e 0+e],c3);plot([0 1 1 0 0],[0 0 1 1 0]);disp('weights');
  "IW{2,1}(642,:)'" : Constant  Value=[-1.2861901654717493581614462527795694768428802490234375;-0.58934198439945639780290775888715870678424835205078125;1.9123452388948212199437648450839333236217498779296875;0.5175482537198903276731698497314937412738800048828125;0.976866912337329917903616660623811185359954833984375;1.5631817963576206675924140654387883841991424560546875;1.2001897932179461658819263902842067182064056396484375;-0.30914959845127587545476899322238750755786895751953125]
      mask Display: e = 0.06;c1 = [120 150 230]/255;c2 = ([120 150 230]+0)/383;c3 = ([120 150 230]+128)/383;patch([0 1 1 0],[0 0 1 1],c1);patch([0 1 1 1-e 1-e 0+e],[0 0 1 1-e 0+e 0+e],c2);patch([0 0 1 1-e 0+e 0+e],[0 1 1 1-e 1-e 0+e],c3);plot([0 1 1 0 0],[0 0 1 1 0]);disp('weights');
  "IW{2,1}(643,:)'" : Constant  Value=[0.1211742012431022974539018832729198038578033447265625;-0.356689297026824114755783057262306101620197296142578125;0.58117137809015739779994191849255003035068511962890625;1.9013816480249356999365772935561835765838623046875;-1.081492553859848992914294285583309829235076904296875;0.58356203222750391290674087940715253353118896484375;1.385146105304001284963533180416561663150787353515625;-1.841638769892946836392866316600702702999114990234375]
      mask Display: e = 0.06;c1 = [120 150 230]/255;c2 = ([120 150 230]+0)/383;c3 = ([120 150 230]+128)/383;patch([0 1 1 0],[0 0 1 1],c1);patch([0 1 1 1-e 1-e 0+e],[0 0 1 1-e 0+e 0+e],c2);patch([0 0 1 1-e 0+e 0+e],[0 1 1 1-e 1-e 0+e],c3);plot([0 1 1 0 0],[0 0 1 1 0]);disp('weights');
  "IW{2,1}(644,:)'" : Constant  Value=[-0.8322971275716042338643774201045744121074676513671875;-1.188587634633992973220983913051895797252655029296875;0.321846647010125497256893822850543074309825897216796875;-1.843223962740573096397156405146233737468719482421875;-0.2148255344487632612082705918510328046977519989013671875;-1.9767754347212116439180817906162701547145843505859375;0.8121184471350610944995196405216120183467864990234375;-0.9020605560629719743559462585835717618465423583984375]
      mask Display: e = 0.06;c1 = [120 150 230]/255;c2 = ([120 150 230]+0)/383;c3 = ([120 150 230]+128)/383;patch([0 1 1 0],[0 0 1 1],c1);patch([0 1 1 1-e 1-e 0+e],[0 0 1 1-e 0+e 0+e],c2);patch([0 0 1 1-e 0+e 0+e],[0 1 1 1-e 1-e 0+e],c3);plot([0 1 1 0 0],[0 0 1 1 0]);disp('weights');
  "IW{2,1}(645,:)'" : Constant  Value=[-1.0341794137452196000737103531719185411930084228515625;-0.92080696102946146819334671818069182336330413818359375;0.405766281627872926751621207586140371859073638916015625;-0.062398168733356081105956292276459862478077411651611328125;-0.5294907842309102274924725861637853085994720458984375;-1.798703539519834748716675676405429840087890625;2.17215194575131231857767488691024482250213623046875;0.9240658204292950816949314685189165174961090087890625]
      mask Display: e = 0.06;c1 = [120 150 230]/255;c2 = ([120 150 230]+0)/383;c3 = ([120 150 230]+128)/383;patch([0 1 1 0],[0 0 1 1],c1);patch([0 1 1 1-e 1-e 0+e],[0 0 1 1-e 0+e 0+e],c2);patch([0 0 1 1-e 0+e 0+e],[0 1 1 1-e 1-e 0+e],c3);plot([0 1 1 0 0],[0 0 1 1 0]);disp('weights');
  "IW{2,1}(646,:)'" : Constant  Value=[1.187026699522312878087859644438140094280242919921875;1.440221883487016185654283617623150348663330078125;1.0482817307158807107470011033001355826854705810546875;-1.029147143200746850055793402134440839290618896484375;1.374836514054156300090880904463119804859161376953125;0.39537133540816526977579314916511066257953643798828125;-1.589786215292808169152749542263336479663848876953125;0.87023060000290997084704258668352849781513214111328125]
      mask Display: e = 0.06;c1 = [120 150 230]/255;c2 = ([120 150 230]+0)/383;c3 = ([120 150 230]+128)/383;patch([0 1 1 0],[0 0 1 1],c1);patch([0 1 1 1-e 1-e 0+e],[0 0 1 1-e 0+e 0+e],c2);patch([0 0 1 1-e 0+e 0+e],[0 1 1 1-e 1-e 0+e],c3);plot([0 1 1 0 0],[0 0 1 1 0]);disp('weights');
  "IW{2,1}(647,:)'" : Constant  Value=[-0.2379308923483981763613570592497126199305057525634765625;0.73587280626997075838602313524461351335048675537109375;0.89351430484891347649778481354587711393833160400390625;-0.307477656034887747438233418506570160388946533203125;0.302899586930296449427402194487513042986392974853515625;-2.342585683593782608369338049669750034809112548828125;1.996742506705442732339861322543583810329437255859375;0.632590361770077880265716885332949459552764892578125]
      mask Display: e = 0.06;c1 = [120 150 230]/255;c2 = ([120 150 230]+0)/383;c3 = ([120 150 230]+128)/383;patch([0 1 1 0],[0 0 1 1],c1);patch([0 1 1 1-e 1-e 0+e],[0 0 1 1-e 0+e 0+e],c2);patch([0 0 1 1-e 0+e 0+e],[0 1 1 1-e 1-e 0+e],c3);plot([0 1 1 0 0],[0 0 1 1 0]);disp('weights');
  "IW{2,1}(648,:)'" : Constant  Value=[-1.92959567361189865408732657670043408870697021484375;-0.09373632972259336726406075968043296597898006439208984375;-0.56506619714617822847202432967606000602245330810546875;-1.4432841128951146014713913245941512286663055419921875;-0.54827621450585850571002310971380211412906646728515625;-1.6857773937402367181448425981216132640838623046875;1.2092212472518628629813974839635193347930908203125;0.53800852735781734548226040715235285460948944091796875]
      mask Display: e = 0.06;c1 = [120 150 230]/255;c2 = ([120 150 230]+0)/383;c3 = ([120 150 230]+128)/383;patch([0 1 1 0],[0 0 1 1],c1);patch([0 1 1 1-e 1-e 0+e],[0 0 1 1-e 0+e 0+e],c2);patch([0 0 1 1-e 0+e 0+e],[0 1 1 1-e 1-e 0+e],c3);plot([0 1 1 0 0],[0 0 1 1 0]);disp('weights');
  "IW{2,1}(649,:)'" : Constant  Value=[1.419290775806361093458463074057362973690032958984375;-1.023520332625797113479393374291248619556427001953125;1.503936103468638929570033724303357303142547607421875;-0.74566808060637412847171390239964239299297332763671875;0.0697691652685075158757399549358524382114410400390625;-1.452303618799362094904381592641584575176239013671875;-1.651431775516365885181357953115366399288177490234375;0.4814444004297246948453903314657509326934814453125]
      mask Display: e = 0.06;c1 = [120 150 230]/255;c2 = ([120 150 230]+0)/383;c3 = ([120 150 230]+128)/383;patch([0 1 1 0],[0 0 1 1],c1);patch([0 1 1 1-e 1-e 0+e],[0 0 1 1-e 0+e 0+e],c2);patch([0 0 1 1-e 0+e 0+e],[0 1 1 1-e 1-e 0+e],c3);plot([0 1 1 0 0],[0 0 1 1 0]);disp('weights');
  "IW{2,1}(65,:)'" : Constant  Value=[-1.973082483605541614934963945415802299976348876953125;-0.2145644422247074689646950673704850487411022186279296875;-1.432957005982654852260793632012791931629180908203125;-0.568642974987701332878486937261186540126800537109375;-2.003227083436929234494527918286621570587158203125;-0.38776796384512068893712921635597012937068939208984375;0.577311998145439542184931269730441272258758544921875;0.57112215390582388163664973035338334739208221435546875]
      mask Display: e = 0.06;c1 = [120 150 230]/255;c2 = ([120 150 230]+0)/383;c3 = ([120 150 230]+128)/383;patch([0 1 1 0],[0 0 1 1],c1);patch([0 1 1 1-e 1-e 0+e],[0 0 1 1-e 0+e 0+e],c2);patch([0 0 1 1-e 0+e 0+e],[0 1 1 1-e 1-e 0+e],c3);plot([0 1 1 0 0],[0 0 1 1 0]);disp('weights');
  "IW{2,1}(650,:)'" : Constant  Value=[-1.8028376363759150979859668950666673481464385986328125;1.0263264862109886532692826222046278417110443115234375;-1.9304766475327383989935015051742084324359893798828125;-0.44938325224649167122237258809036575257778167724609375;0.5433279106748312159425040590576827526092529296875;-0.30516726343965128176449752572807483375072479248046875;1.255951845611958272996844243607483804225921630859375;0.99844815025894850801790880723274312913417816162109375]
      mask Display: e = 0.06;c1 = [120 150 230]/255;c2 = ([120 150 230]+0)/383;c3 = ([120 150 230]+128)/383;patch([0 1 1 0],[0 0 1 1],c1);patch([0 1 1 1-e 1-e 0+e],[0 0 1 1-e 0+e 0+e],c2);patch([0 0 1 1-e 0+e 0+e],[0 1 1 1-e 1-e 0+e],c3);plot([0 1 1 0 0],[0 0 1 1 0]);disp('weights');
  "IW{2,1}(651,:)'" : Constant  Value=[-0.8800613073923617690752507769502699375152587890625;-1.022353287914410824299693558714352548122406005859375;1.616135649662293172212912395480088889598846435546875;-0.400501305535721219275302473761257715523242950439453125;-1.70110401953730416835242067463696002960205078125;0.640993310445694408628014571149833500385284423828125;-1.6182951378719436785758034602622501552104949951171875;-0.7305551235819820465877683091093786060810089111328125]
      mask Display: e = 0.06;c1 = [120 150 230]/255;c2 = ([120 150 230]+0)/383;c3 = ([120 150 230]+128)/383;patch([0 1 1 0],[0 0 1 1],c1);patch([0 1 1 1-e 1-e 0+e],[0 0 1 1-e 0+e 0+e],c2);patch([0 0 1 1-e 0+e 0+e],[0 1 1 1-e 1-e 0+e],c3);plot([0 1 1 0 0],[0 0 1 1 0]);disp('weights');
  "IW{2,1}(652,:)'" : Constant  Value=[1.477217814075697077669246937148272991180419921875;-1.55736145948020432427938430919311940670013427734375;1.5577505509069651257192390403361059725284576416015625;0.63516240999488282614748868581955321133136749267578125;-0.55422529926720975890219733628327958285808563232421875;-1.7098574804653667857934351559379138052463531494140625;0.3410931369338694452153504244051873683929443359375;0.302708089613833275510756948278867639601230621337890625]
      mask Display: e = 0.06;c1 = [120 150 230]/255;c2 = ([120 150 230]+0)/383;c3 = ([120 150 230]+128)/383;patch([0 1 1 0],[0 0 1 1],c1);patch([0 1 1 1-e 1-e 0+e],[0 0 1 1-e 0+e 0+e],c2);patch([0 0 1 1-e 0+e 0+e],[0 1 1 1-e 1-e 0+e],c3);plot([0 1 1 0 0],[0 0 1 1 0]);disp('weights');
  "IW{2,1}(653,:)'" : Constant  Value=[-1.5873072364539011491757491967291571199893951416015625;0.52866897960869241313019983863341622054576873779296875;-0.74175830385214125417547847973764874041080474853515625;-0.11959613769250233838992159007830196060240268707275390625;0.361396597656525653263770436751656234264373779296875;1.5330012603949672023162520417827181518077850341796875;-2.24437423766952282022657527704723179340362548828125;0.3799233096749679017278822357184253633022308349609375]
      mask Display: e = 0.06;c1 = [120 150 230]/255;c2 = ([120 150 230]+0)/383;c3 = ([120 150 230]+128)/383;patch([0 1 1 0],[0 0 1 1],c1);patch([0 1 1 1-e 1-e 0+e],[0 0 1 1-e 0+e 0+e],c2);patch([0 0 1 1-e 0+e 0+e],[0 1 1 1-e 1-e 0+e],c3);plot([0 1 1 0 0],[0 0 1 1 0]);disp('weights');
  "IW{2,1}(654,:)'" : Constant  Value=[-0.455323341881275711617860224578180350363254547119140625;-0.5841949407720667952759185936884023249149322509765625;0.7413358341625702063737435310031287372112274169921875;-0.5760132713601893161836642320849932730197906494140625;-2.0909975359619199508642850560136139392852783203125;0.0542959667542441681842291245629894547164440155029296875;-2.275357540657048982524202074273489415645599365234375;0.1723428942532114482855121195825631730258464813232421875]
      mask Display: e = 0.06;c1 = [120 150 230]/255;c2 = ([120 150 230]+0)/383;c3 = ([120 150 230]+128)/383;patch([0 1 1 0],[0 0 1 1],c1);patch([0 1 1 1-e 1-e 0+e],[0 0 1 1-e 0+e 0+e],c2);patch([0 0 1 1-e 0+e 0+e],[0 1 1 1-e 1-e 0+e],c3);plot([0 1 1 0 0],[0 0 1 1 0]);disp('weights');
  "IW{2,1}(655,:)'" : Constant  Value=[-0.9273958360241201237528230194584466516971588134765625;-1.6294807970735278868090745163499377667903900146484375;1.4883391922949076313642535751569084823131561279296875;-1.794674354340346500435998677858151495456695556640625;-0.391439730933659302269944646468502469360828399658203125;-0.307844723325147617831731849946663714945316314697265625;-0.1974153419941396536696487373774289153516292572021484375;1.3158527444748637780236322214477695524692535400390625]
      mask Display: e = 0.06;c1 = [120 150 230]/255;c2 = ([120 150 230]+0)/383;c3 = ([120 150 230]+128)/383;patch([0 1 1 0],[0 0 1 1],c1);patch([0 1 1 1-e 1-e 0+e],[0 0 1 1-e 0+e 0+e],c2);patch([0 0 1 1-e 0+e 0+e],[0 1 1 1-e 1-e 0+e],c3);plot([0 1 1 0 0],[0 0 1 1 0]);disp('weights');
  "IW{2,1}(656,:)'" : Constant  Value=[1.7973910861721911214061719874734990298748016357421875;1.176207486113776123914931304170750081539154052734375;-0.159975251502850301932312504504807293415069580078125;1.27598425405775106611372393672354519367218017578125;0.93024919495184821283118026258307509124279022216796875;0.2185534130075611758403653084315010346472263336181640625;0.9690586139220318528941788827069103717803955078125;-1.6970762795498568475949241474154405295848846435546875]
      mask Display: e = 0.06;c1 = [120 150 230]/255;c2 = ([120 150 230]+0)/383;c3 = ([120 150 230]+128)/383;patch([0 1 1 0],[0 0 1 1],c1);patch([0 1 1 1-e 1-e 0+e],[0 0 1 1-e 0+e 0+e],c2);patch([0 0 1 1-e 0+e 0+e],[0 1 1 1-e 1-e 0+e],c3);plot([0 1 1 0 0],[0 0 1 1 0]);disp('weights');
  "IW{2,1}(657,:)'" : Constant  Value=[1.632732071243712113073343061842024326324462890625;0.017028793649021954637046150082824169658124446868896484375;-1.0547591410428349689709648373536765575408935546875;0.7678145404622487291135257692076265811920166015625;-1.5022660310973019459623856164398603141307830810546875;1.614987899846425545291594971786253154277801513671875;0.4485040268382378680911415358423255383968353271484375;1.2542554606795164318100432865321636199951171875]
      mask Display: e = 0.06;c1 = [120 150 230]/255;c2 = ([120 150 230]+0)/383;c3 = ([120 150 230]+128)/383;patch([0 1 1 0],[0 0 1 1],c1);patch([0 1 1 1-e 1-e 0+e],[0 0 1 1-e 0+e 0+e],c2);patch([0 0 1 1-e 0+e 0+e],[0 1 1 1-e 1-e 0+e],c3);plot([0 1 1 0 0],[0 0 1 1 0]);disp('weights');
  "IW{2,1}(658,:)'" : Constant  Value=[1.898335204141020415846696778316982090473175048828125;-0.1681759071121402826509694250489701516926288604736328125;0.7770597868535780161636239427025429904460906982421875;0.0576122973361552770388271937918034382164478302001953125;1.4827302646230295923857056550332345068454742431640625;1.00507928229243770346101882751099765300750732421875;-1.8773419364391799035729491151869297027587890625;0.0003042913359580534139736673893139595747925341129302978515625]
      mask Display: e = 0.06;c1 = [120 150 230]/255;c2 = ([120 150 230]+0)/383;c3 = ([120 150 230]+128)/383;patch([0 1 1 0],[0 0 1 1],c1);patch([0 1 1 1-e 1-e 0+e],[0 0 1 1-e 0+e 0+e],c2);patch([0 0 1 1-e 0+e 0+e],[0 1 1 1-e 1-e 0+e],c3);plot([0 1 1 0 0],[0 0 1 1 0]);disp('weights');
  "IW{2,1}(659,:)'" : Constant  Value=[1.305114095815213648421604375471360981464385986328125;-1.085711833302984263838197875884361565113067626953125;-0.76126542311254874473291920367046259343624114990234375;-1.0833352518673311504215917011606507003307342529296875;1.6180690177445697930380674733896739780902862548828125;1.5447962665866008524773178578470833599567413330078125;0.70373727971780819512304105955990962684154510498046875;0.93883349411831085173929523080005310475826263427734375]
      mask Display: e = 0.06;c1 = [120 150 230]/255;c2 = ([120 150 230]+0)/383;c3 = ([120 150 230]+128)/383;patch([0 1 1 0],[0 0 1 1],c1);patch([0 1 1 1-e 1-e 0+e],[0 0 1 1-e 0+e 0+e],c2);patch([0 0 1 1-e 0+e 0+e],[0 1 1 1-e 1-e 0+e],c3);plot([0 1 1 0 0],[0 0 1 1 0]);disp('weights');
  "IW{2,1}(66,:)'" : Constant  Value=[-0.09341247792529398796812500904707121662795543670654296875;0.266183777289563938683869537271675653755664825439453125;0.7248788409664561616096989382640458643436431884765625;-2.214528714173861434488799204700626432895660400390625;-1.528111460753998951389576177462004125118255615234375;-0.75937514408108197638824776731780730187892913818359375;1.0653444866019741166240919483243487775325775146484375;-1.0954715249246422814621837460435926914215087890625]
      mask Display: e = 0.06;c1 = [120 150 230]/255;c2 = ([120 150 230]+0)/383;c3 = ([120 150 230]+128)/383;patch([0 1 1 0],[0 0 1 1],c1);patch([0 1 1 1-e 1-e 0+e],[0 0 1 1-e 0+e 0+e],c2);patch([0 0 1 1-e 0+e 0+e],[0 1 1 1-e 1-e 0+e],c3);plot([0 1 1 0 0],[0 0 1 1 0]);disp('weights');
  "IW{2,1}(660,:)'" : Constant  Value=[-0.68225531774445913324456114423810504376888275146484375;1.4332893299764870587154064196511171758174896240234375;-1.461936035818782730899556554504670202732086181640625;-0.31573108566166585564616298142937012016773223876953125;-1.8317446436653705976738137906068004667758941650390625;0.74760604755668869092488648675498552620410919189453125;-1.348625760055722988539628204307518899440765380859375;0.72092270911420452961237970157526433467864990234375]
      mask Display: e = 0.06;c1 = [120 150 230]/255;c2 = ([120 150 230]+0)/383;c3 = ([120 150 230]+128)/383;patch([0 1 1 0],[0 0 1 1],c1);patch([0 1 1 1-e 1-e 0+e],[0 0 1 1-e 0+e 0+e],c2);patch([0 0 1 1-e 0+e 0+e],[0 1 1 1-e 1-e 0+e],c3);plot([0 1 1 0 0],[0 0 1 1 0]);disp('weights');
  "IW{2,1}(661,:)'" : Constant  Value=[0.92421304714781260525313655307400040328502655029296875;-1.9349253006059032866659208593773655593395233154296875;-1.8533325572209751186392168165184557437896728515625;0.06697932875211794201408821436416474170982837677001953125;0.199282188740755039635388357055489905178546905517578125;-0.86832684857009978518505022293538786470890045166015625;-1.29058242990658644799850662820972502231597900390625;0.520258794344968134026885309140197932720184326171875]
      mask Display: e = 0.06;c1 = [120 150 230]/255;c2 = ([120 150 230]+0)/383;c3 = ([120 150 230]+128)/383;patch([0 1 1 0],[0 0 1 1],c1);patch([0 1 1 1-e 1-e 0+e],[0 0 1 1-e 0+e 0+e],c2);patch([0 0 1 1-e 0+e 0+e],[0 1 1 1-e 1-e 0+e],c3);plot([0 1 1 0 0],[0 0 1 1 0]);disp('weights');
  "IW{2,1}(662,:)'" : Constant  Value=[1.5821282256354629591754701323225162923336029052734375;-1.5428486351814052479625161140575073659420013427734375;1.3664912755442297775942961379769258201122283935546875;-0.094764707002653103540268375581945292651653289794921875;0.9227196720302848209627200048998929560184478759765625;1.3825614945692941137878051449661143124103546142578125;-0.77150900648655429403532934884424321353435516357421875;-1.00223033266867478374706479371525347232818603515625]
      mask Display: e = 0.06;c1 = [120 150 230]/255;c2 = ([120 150 230]+0)/383;c3 = ([120 150 230]+128)/383;patch([0 1 1 0],[0 0 1 1],c1);patch([0 1 1 1-e 1-e 0+e],[0 0 1 1-e 0+e 0+e],c2);patch([0 0 1 1-e 0+e 0+e],[0 1 1 1-e 1-e 0+e],c3);plot([0 1 1 0 0],[0 0 1 1 0]);disp('weights');
  "IW{2,1}(663,:)'" : Constant  Value=[-0.9534966131388660226519959905999712646007537841796875;-1.1836160531979686982850807908107526600360870361328125;1.3908003420912466996384182493784464895725250244140625;-1.8092776466909710197938920828164555132389068603515625;-0.0261278934148914711299571678182473988272249698638916015625;-1.1821983856247648692061602559988386929035186767578125;-0.463372509060189063934132036592927761375904083251953125;1.3585578025746529728934319791733287274837493896484375]
      mask Display: e = 0.06;c1 = [120 150 230]/255;c2 = ([120 150 230]+0)/383;c3 = ([120 150 230]+128)/383;patch([0 1 1 0],[0 0 1 1],c1);patch([0 1 1 1-e 1-e 0+e],[0 0 1 1-e 0+e 0+e],c2);patch([0 0 1 1-e 0+e 0+e],[0 1 1 1-e 1-e 0+e],c3);plot([0 1 1 0 0],[0 0 1 1 0]);disp('weights');
  "IW{2,1}(664,:)'" : Constant  Value=[-1.950458050173903945534448212129063904285430908203125;0.86937083519382241103556907546590082347393035888671875;1.1428698553688061423372346325777471065521240234375;-0.648356106539008436584481387399137020111083984375;-0.1592394147138106175187743929200223647058010101318359375;1.5225565534273755030625352446804754436016082763671875;-0.57832621788909743809625751964631490409374237060546875;-1.4752198616116094509465028750128112733364105224609375]
      mask Display: e = 0.06;c1 = [120 150 230]/255;c2 = ([120 150 230]+0)/383;c3 = ([120 150 230]+128)/383;patch([0 1 1 0],[0 0 1 1],c1);patch([0 1 1 1-e 1-e 0+e],[0 0 1 1-e 0+e 0+e],c2);patch([0 0 1 1-e 0+e 0+e],[0 1 1 1-e 1-e 0+e],c3);plot([0 1 1 0 0],[0 0 1 1 0]);disp('weights');
  "IW{2,1}(665,:)'" : Constant  Value=[-1.1476693837524891694812367859412916004657745361328125;-1.538776705651164089516669264412485063076019287109375;-1.63714922238856441794041529647074639797210693359375;-1.55638064756071781147284127655439078807830810546875;-0.302232886428215719032408514976850710809230804443359375;-0.56657431029165905567168692869017831981182098388671875;0.768650812566308072604215340106748044490814208984375;1.1259517975457067340272487854235805571079254150390625]
      mask Display: e = 0.06;c1 = [120 150 230]/255;c2 = ([120 150 230]+0)/383;c3 = ([120 150 230]+128)/383;patch([0 1 1 0],[0 0 1 1],c1);patch([0 1 1 1-e 1-e 0+e],[0 0 1 1-e 0+e 0+e],c2);patch([0 0 1 1-e 0+e 0+e],[0 1 1 1-e 1-e 0+e],c3);plot([0 1 1 0 0],[0 0 1 1 0]);disp('weights');
  "IW{2,1}(666,:)'" : Constant  Value=[-0.95313530152680525642239217631868086755275726318359375;-1.6787003651176355401020146018709056079387664794921875;1.164266943076947224966488647623918950557708740234375;-0.60560094681233522795338330979575403034687042236328125;-1.0722082257728551279996054290677420794963836669921875;-0.88546617467856825189898017924861051142215728759765625;1.7530311144628425434888185918680392205715179443359375;0.67673973579510915410395455182879231870174407958984375]
      mask Display: e = 0.06;c1 = [120 150 230]/255;c2 = ([120 150 230]+0)/383;c3 = ([120 150 230]+128)/383;patch([0 1 1 0],[0 0 1 1],c1);patch([0 1 1 1-e 1-e 0+e],[0 0 1 1-e 0+e 0+e],c2);patch([0 0 1 1-e 0+e 0+e],[0 1 1 1-e 1-e 0+e],c3);plot([0 1 1 0 0],[0 0 1 1 0]);disp('weights');
  "IW{2,1}(667,:)'" : Constant  Value=[-1.1023422502967263891804350350867025554180145263671875;1.461280617070430221104970769374631345272064208984375;0.166672768832424045282181168659008108079433441162109375;-1.83822883852159701945083725149743258953094482421875;1.2120464046259431523111516071367077529430389404296875;-1.14988069955171567926299758255481719970703125;-0.046763039703135882152462698968520271591842174530029296875;-1.265254437567301604161684736027382314205169677734375]
      mask Display: e = 0.06;c1 = [120 150 230]/255;c2 = ([120 150 230]+0)/383;c3 = ([120 150 230]+128)/383;patch([0 1 1 0],[0 0 1 1],c1);patch([0 1 1 1-e 1-e 0+e],[0 0 1 1-e 0+e 0+e],c2);patch([0 0 1 1-e 0+e 0+e],[0 1 1 1-e 1-e 0+e],c3);plot([0 1 1 0 0],[0 0 1 1 0]);disp('weights');
  "IW{2,1}(668,:)'" : Constant  Value=[-2.04143060862283931555793969891965389251708984375;-0.0224101600513481706566931705992828938178718090057373046875;-0.12162567786143245462948669910474563948810100555419921875;1.1236450167381624165585662922239862382411956787109375;0.075437972333445013628505648739519529044628143310546875;-1.9515445946950766842320490468409843742847442626953125;0.035121906052087946414896890701129450462758541107177734375;-1.3462080092698183175770054731401614844799041748046875]
      mask Display: e = 0.06;c1 = [120 150 230]/255;c2 = ([120 150 230]+0)/383;c3 = ([120 150 230]+128)/383;patch([0 1 1 0],[0 0 1 1],c1);patch([0 1 1 1-e 1-e 0+e],[0 0 1 1-e 0+e 0+e],c2);patch([0 0 1 1-e 0+e 0+e],[0 1 1 1-e 1-e 0+e],c3);plot([0 1 1 0 0],[0 0 1 1 0]);disp('weights');
  "IW{2,1}(669,:)'" : Constant  Value=[0.99448271823922784751204062558826990425586700439453125;-0.147382310612668210314524230852839536964893341064453125;-0.60924203484304217948164250628906302154064178466796875;1.5696497545588334876498493031249381601810455322265625;1.3802442087894213340604210316087119281291961669921875;-1.6712682061764116969726501338300295174121856689453125;-0.829640378764258112909146802849136292934417724609375;-1.4237769199087033644701705270563252270221710205078125]
      mask Display: e = 0.06;c1 = [120 150 230]/255;c2 = ([120 150 230]+0)/383;c3 = ([120 150 230]+128)/383;patch([0 1 1 0],[0 0 1 1],c1);patch([0 1 1 1-e 1-e 0+e],[0 0 1 1-e 0+e 0+e],c2);patch([0 0 1 1-e 0+e 0+e],[0 1 1 1-e 1-e 0+e],c3);plot([0 1 1 0 0],[0 0 1 1 0]);disp('weights');
  "IW{2,1}(67,:)'" : Constant  Value=[-0.264021076503246854283446509725763462483882904052734375;-0.79829733773377287153749648496159352362155914306640625;-0.41966867095028426160041590264881961047649383544921875;0.66893618850172120726682578606414608657360076904296875;0.06713199748941640898625138333954964764416217803955078125;1.9939545064037751398444697770173661410808563232421875;-2.227108853697944201854852508404292166233062744140625;-0.70299155655797651576222051517106592655181884765625]
      mask Display: e = 0.06;c1 = [120 150 230]/255;c2 = ([120 150 230]+0)/383;c3 = ([120 150 230]+128)/383;patch([0 1 1 0],[0 0 1 1],c1);patch([0 1 1 1-e 1-e 0+e],[0 0 1 1-e 0+e 0+e],c2);patch([0 0 1 1-e 0+e 0+e],[0 1 1 1-e 1-e 0+e],c3);plot([0 1 1 0 0],[0 0 1 1 0]);disp('weights');
  "IW{2,1}(670,:)'" : Constant  Value=[1.683432089134687448250815577921457588672637939453125;1.0778149123355833527426739237853325903415679931640625;1.672378506448554791319338619359768927097320556640625;-0.7242401871731642959417740712524391710758209228515625;1.35583214012320052432869488256983458995819091796875;0.71413676019540750505854020957485772669315338134765625;0.27715612613140461206739928456954658031463623046875;1.133699630854529072365721731330268085002899169921875]
      mask Display: e = 0.06;c1 = [120 150 230]/255;c2 = ([120 150 230]+0)/383;c3 = ([120 150 230]+128)/383;patch([0 1 1 0],[0 0 1 1],c1);patch([0 1 1 1-e 1-e 0+e],[0 0 1 1-e 0+e 0+e],c2);patch([0 0 1 1-e 0+e 0+e],[0 1 1 1-e 1-e 0+e],c3);plot([0 1 1 0 0],[0 0 1 1 0]);disp('weights');
  "IW{2,1}(671,:)'" : Constant  Value=[1.4997050432369773975693760803551413118839263916015625;0.007115681224748261236856539113659891881980001926422119140625;0.864423294920222407000665043597109615802764892578125;-1.621343424800654187123427618644200265407562255859375;-0.07380011352077460451415191755586420185863971710205078125;1.424946783616969359087534030550159513950347900390625;-1.0391119455601300902714001495041884481906890869140625;1.5222445664897801265169619000516831874847412109375]
      mask Display: e = 0.06;c1 = [120 150 230]/255;c2 = ([120 150 230]+0)/383;c3 = ([120 150 230]+128)/383;patch([0 1 1 0],[0 0 1 1],c1);patch([0 1 1 1-e 1-e 0+e],[0 0 1 1-e 0+e 0+e],c2);patch([0 0 1 1-e 0+e 0+e],[0 1 1 1-e 1-e 0+e],c3);plot([0 1 1 0 0],[0 0 1 1 0]);disp('weights');
  "IW{2,1}(672,:)'" : Constant  Value=[1.2893214660036027563450033994740806519985198974609375;0.2175689424429260998561375117787974886596202850341796875;-1.5541424342787097945262075882055796682834625244140625;-1.1058195831665302844015741356997750699520111083984375;0.90526333232334099676563710090704262256622314453125;-0.39470628538045715583137962312321178615093231201171875;2.02702372321686130618445531581528484821319580078125;-0.782432869623763682653816431411541998386383056640625]
      mask Display: e = 0.06;c1 = [120 150 230]/255;c2 = ([120 150 230]+0)/383;c3 = ([120 150 230]+128)/383;patch([0 1 1 0],[0 0 1 1],c1);patch([0 1 1 1-e 1-e 0+e],[0 0 1 1-e 0+e 0+e],c2);patch([0 0 1 1-e 0+e 0+e],[0 1 1 1-e 1-e 0+e],c3);plot([0 1 1 0 0],[0 0 1 1 0]);disp('weights');
  "IW{2,1}(673,:)'" : Constant  Value=[1.8109683572609209800674534562858752906322479248046875;0.677613783411000536460733201238326728343963623046875;0.225287245137875735689902967351372353732585906982421875;-1.356365146687422029714298332692123949527740478515625;0.56266885218466822227156853841734118759632110595703125;1.456458924196455395616567329852841794490814208984375;1.58967287232168796862197268637828528881072998046875;-0.64617101704868240563683912114356644451618194580078125]
      mask Display: e = 0.06;c1 = [120 150 230]/255;c2 = ([120 150 230]+0)/383;c3 = ([120 150 230]+128)/383;patch([0 1 1 0],[0 0 1 1],c1);patch([0 1 1 1-e 1-e 0+e],[0 0 1 1-e 0+e 0+e],c2);patch([0 0 1 1-e 0+e 0+e],[0 1 1 1-e 1-e 0+e],c3);plot([0 1 1 0 0],[0 0 1 1 0]);disp('weights');
  "IW{2,1}(674,:)'" : Constant  Value=[-0.95258819522533821899656913956278003752231597900390625;-1.25744550122118514678959400043822824954986572265625;0.80723741622791600480724127919529564678668975830078125;1.995748592621650718825776493758894503116607666015625;-1.7108407601099837602731668084743432700634002685546875;-0.64969041269219196532702653712476603686809539794921875;-0.76484115310527378550631283360417000949382781982421875;0.050586150390545030208766519308483111672103404998779296875]
      mask Display: e = 0.06;c1 = [120 150 230]/255;c2 = ([120 150 230]+0)/383;c3 = ([120 150 230]+128)/383;patch([0 1 1 0],[0 0 1 1],c1);patch([0 1 1 1-e 1-e 0+e],[0 0 1 1-e 0+e 0+e],c2);patch([0 0 1 1-e 0+e 0+e],[0 1 1 1-e 1-e 0+e],c3);plot([0 1 1 0 0],[0 0 1 1 0]);disp('weights');
  "IW{2,1}(675,:)'" : Constant  Value=[-0.0788641968398575421428375875620986334979534149169921875;0.0935950590999269083081202325047343038022518157958984375;-0.651439766033151013147062258212827146053314208984375;-1.664629932502772025060266969376243650913238525390625;-1.738532712945103586577033638604916632175445556640625;-1.219585429891332228891087652300484478473663330078125;-1.81281235005932739312584089930169284343719482421875;-0.13418464067722524202252998293261043727397918701171875]
      mask Display: e = 0.06;c1 = [120 150 230]/255;c2 = ([120 150 230]+0)/383;c3 = ([120 150 230]+128)/383;patch([0 1 1 0],[0 0 1 1],c1);patch([0 1 1 1-e 1-e 0+e],[0 0 1 1-e 0+e 0+e],c2);patch([0 0 1 1-e 0+e 0+e],[0 1 1 1-e 1-e 0+e],c3);plot([0 1 1 0 0],[0 0 1 1 0]);disp('weights');
  "IW{2,1}(676,:)'" : Constant  Value=[-1.1218265877348707615368539336486719548702239990234375;1.6337574819893954103378064246498979628086090087890625;-1.5773391083701417958451429512933827936649322509765625;-0.410677925744585003986486526628141291439533233642578125;1.131443277581542616871956852264702320098876953125;-1.3252139200527086604353144139167852699756622314453125;-0.469814981713228052573327886420884169638156890869140625;-1.066138992155289511032378868549130856990814208984375]
      mask Display: e = 0.06;c1 = [120 150 230]/255;c2 = ([120 150 230]+0)/383;c3 = ([120 150 230]+128)/383;patch([0 1 1 0],[0 0 1 1],c1);patch([0 1 1 1-e 1-e 0+e],[0 0 1 1-e 0+e 0+e],c2);patch([0 0 1 1-e 0+e 0+e],[0 1 1 1-e 1-e 0+e],c3);plot([0 1 1 0 0],[0 0 1 1 0]);disp('weights');
  "IW{2,1}(677,:)'" : Constant  Value=[0.77139593928472560691034232149831950664520263671875;-1.1757086594908947585480518682743422687053680419921875;-0.5338452151382859778294687203015200793743133544921875;1.9352815130630809381528933954541571438312530517578125;0.89046368795363151082966624016989953815937042236328125;1.71608004327114560538802834344096481800079345703125;0.0786435936999058948781993194643291644752025604248046875;-1.14076491905498134116214714595116674900054931640625]
      mask Display: e = 0.06;c1 = [120 150 230]/255;c2 = ([120 150 230]+0)/383;c3 = ([120 150 230]+128)/383;patch([0 1 1 0],[0 0 1 1],c1);patch([0 1 1 1-e 1-e 0+e],[0 0 1 1-e 0+e 0+e],c2);patch([0 0 1 1-e 0+e 0+e],[0 1 1 1-e 1-e 0+e],c3);plot([0 1 1 0 0],[0 0 1 1 0]);disp('weights');
  "IW{2,1}(678,:)'" : Constant  Value=[-1.5375576375621962110784579635947011411190032958984375;0.308871908588343180301905022133723832666873931884765625;0.43609617748450391072623233412741683423519134521484375;1.2365360837277921124410795528092421591281890869140625;1.621500759825130533187120818183757364749908447265625;-1.4790398560006068340300089403172023594379425048828125;1.134439346117375180256203748285770416259765625;0.65875578199072404306235739568364806473255157470703125]
      mask Display: e = 0.06;c1 = [120 150 230]/255;c2 = ([120 150 230]+0)/383;c3 = ([120 150 230]+128)/383;patch([0 1 1 0],[0 0 1 1],c1);patch([0 1 1 1-e 1-e 0+e],[0 0 1 1-e 0+e 0+e],c2);patch([0 0 1 1-e 0+e 0+e],[0 1 1 1-e 1-e 0+e],c3);plot([0 1 1 0 0],[0 0 1 1 0]);disp('weights');
  "IW{2,1}(679,:)'" : Constant  Value=[1.1294081489551661690029504825361073017120361328125;1.7027041718673034953468459207215346395969390869140625;1.4018084951656017977938972762785851955413818359375;0.55551549753475637505317763498169369995594024658203125;1.025005180982395014410712974495254456996917724609375;-0.9171881259677825415366214656387455761432647705078125;-1.6187288447429473148275747007573954761028289794921875;0.2280898139292304171998893025374854914844036102294921875]
      mask Display: e = 0.06;c1 = [120 150 230]/255;c2 = ([120 150 230]+0)/383;c3 = ([120 150 230]+128)/383;patch([0 1 1 0],[0 0 1 1],c1);patch([0 1 1 1-e 1-e 0+e],[0 0 1 1-e 0+e 0+e],c2);patch([0 0 1 1-e 0+e 0+e],[0 1 1 1-e 1-e 0+e],c3);plot([0 1 1 0 0],[0 0 1 1 0]);disp('weights');
  "IW{2,1}(68,:)'" : Constant  Value=[-1.6270702038559907709469598557916469871997833251953125;-1.0261114903483770088854498681030236184597015380859375;-0.653112498864379720231454484746791422367095947265625;-1.6626900076181987397916373083717189729213714599609375;0.88863256726536998808541056860121898353099822998046875;-1.207519594459927514407127091544680297374725341796875;1.0053122528912066258044433197937905788421630859375;-0.98387589531695252009768637435627169907093048095703125]
      mask Display: e = 0.06;c1 = [120 150 230]/255;c2 = ([120 150 230]+0)/383;c3 = ([120 150 230]+128)/383;patch([0 1 1 0],[0 0 1 1],c1);patch([0 1 1 1-e 1-e 0+e],[0 0 1 1-e 0+e 0+e],c2);patch([0 0 1 1-e 0+e 0+e],[0 1 1 1-e 1-e 0+e],c3);plot([0 1 1 0 0],[0 0 1 1 0]);disp('weights');
  "IW{2,1}(680,:)'" : Constant  Value=[0.539949085339345824507972793071530759334564208984375;1.7361881960695264570659901437466032803058624267578125;-0.99089942452622958857233470553182996809482574462890625;-1.251261506362689512883434872492216527462005615234375;0.41018812872337573338654692634008824825286865234375;0.59181000388886595420245839704875834286212921142578125;-1.5703041650046591914957616609171964228153228759765625;1.4574640578132183055259929460589773952960968017578125]
      mask Display: e = 0.06;c1 = [120 150 230]/255;c2 = ([120 150 230]+0)/383;c3 = ([120 150 230]+128)/383;patch([0 1 1 0],[0 0 1 1],c1);patch([0 1 1 1-e 1-e 0+e],[0 0 1 1-e 0+e 0+e],c2);patch([0 0 1 1-e 0+e 0+e],[0 1 1 1-e 1-e 0+e],c3);plot([0 1 1 0 0],[0 0 1 1 0]);disp('weights');
  "IW{2,1}(681,:)'" : Constant  Value=[1.5171825155395388673440493221278302371501922607421875;0.5833714369438369740095140514313243329524993896484375;-0.91241413115811165202018173658871091902256011962890625;-1.0764578391054462347398157362476922571659088134765625;-1.6715294058015859324228813420631922781467437744140625;-1.43379431052576844507484565838240087032318115234375;0.35560284617388571160034871354582719504833221435546875;-1.22877508563357906723467749543488025665283203125]
      mask Display: e = 0.06;c1 = [120 150 230]/255;c2 = ([120 150 230]+0)/383;c3 = ([120 150 230]+128)/383;patch([0 1 1 0],[0 0 1 1],c1);patch([0 1 1 1-e 1-e 0+e],[0 0 1 1-e 0+e 0+e],c2);patch([0 0 1 1-e 0+e 0+e],[0 1 1 1-e 1-e 0+e],c3);plot([0 1 1 0 0],[0 0 1 1 0]);disp('weights');
  "IW{2,1}(682,:)'" : Constant  Value=[-0.455124881041288620320273139441269449889659881591796875;0.72545780585794250594489085415261797606945037841796875;-1.604265715413340398498576178099028766155242919921875;-1.3680816522599579254659829530282877385616302490234375;1.0715069233823946159844808789785020053386688232421875;1.6291913725721105521415665862150490283966064453125;0.499948502829458074625534891310962848365306854248046875;-1.2367851152375008982886583908111788332462310791015625]
      mask Display: e = 0.06;c1 = [120 150 230]/255;c2 = ([120 150 230]+0)/383;c3 = ([120 150 230]+128)/383;patch([0 1 1 0],[0 0 1 1],c1);patch([0 1 1 1-e 1-e 0+e],[0 0 1 1-e 0+e 0+e],c2);patch([0 0 1 1-e 0+e 0+e],[0 1 1 1-e 1-e 0+e],c3);plot([0 1 1 0 0],[0 0 1 1 0]);disp('weights');
  "IW{2,1}(683,:)'" : Constant  Value=[-0.9606534373706414609017656403011642396450042724609375;-1.6210625782737004829670013350551016628742218017578125;0.465942808784856887793779378625913523137569427490234375;1.443621920149970261348926214850507676601409912109375;1.020014770569904527519611292518675327301025390625;-0.76035789762212779852035282601718790829181671142578125;-1.712312920412092154265337740071117877960205078125;-0.76283181323886106728338063476257957518100738525390625]
      mask Display: e = 0.06;c1 = [120 150 230]/255;c2 = ([120 150 230]+0)/383;c3 = ([120 150 230]+128)/383;patch([0 1 1 0],[0 0 1 1],c1);patch([0 1 1 1-e 1-e 0+e],[0 0 1 1-e 0+e 0+e],c2);patch([0 0 1 1-e 0+e 0+e],[0 1 1 1-e 1-e 0+e],c3);plot([0 1 1 0 0],[0 0 1 1 0]);disp('weights');
  "IW{2,1}(684,:)'" : Constant  Value=[0.8012792577753184986022461089305579662322998046875;1.6178059149556249796120255268760956823825836181640625;-0.58666831691273946258746718740439973771572113037109375;1.4827053834778503027536089575733058154582977294921875;-1.2244299657924966329147764554363675415515899658203125;1.6311744323421020208542131513240747153759002685546875;1.00883359717099008179275188012979924678802490234375;0.10450159391982845324964301880754646845161914825439453125]
      mask Display: e = 0.06;c1 = [120 150 230]/255;c2 = ([120 150 230]+0)/383;c3 = ([120 150 230]+128)/383;patch([0 1 1 0],[0 0 1 1],c1);patch([0 1 1 1-e 1-e 0+e],[0 0 1 1-e 0+e 0+e],c2);patch([0 0 1 1-e 0+e 0+e],[0 1 1 1-e 1-e 0+e],c3);plot([0 1 1 0 0],[0 0 1 1 0]);disp('weights');
  "IW{2,1}(685,:)'" : Constant  Value=[-0.271142275312253377972382395455497317016124725341796875;-0.669109512146545792887764037004671990871429443359375;-0.52436954063011731452803587671951390802860260009765625;-1.3931178012409393129900081476080231368541717529296875;2.3521406024869886408623642637394368648529052734375;0.33217197604692838552864486700855195522308349609375;-0.440296170894660277017607086236239410936832427978515625;-1.500906544408965093140295721241272985935211181640625]
      mask Display: e = 0.06;c1 = [120 150 230]/255;c2 = ([120 150 230]+0)/383;c3 = ([120 150 230]+128)/383;patch([0 1 1 0],[0 0 1 1],c1);patch([0 1 1 1-e 1-e 0+e],[0 0 1 1-e 0+e 0+e],c2);patch([0 0 1 1-e 0+e 0+e],[0 1 1 1-e 1-e 0+e],c3);plot([0 1 1 0 0],[0 0 1 1 0]);disp('weights');
  "IW{2,1}(686,:)'" : Constant  Value=[0.8759331690243465917689036359661258757114410400390625;-0.8633401491336822886069057858549058437347412109375;-0.810096131668496699518300374620594084262847900390625;-1.868931012288685966638013269403018057346343994140625;-1.1832092205993987032996983543853275477886199951171875;0.1503251611498417072976252484295400790870189666748046875;-1.94334715604842056535517258453182876110076904296875;-0.353420372878824384788032375581678934395313262939453125]
      mask Display: e = 0.06;c1 = [120 150 230]/255;c2 = ([120 150 230]+0)/383;c3 = ([120 150 230]+128)/383;patch([0 1 1 0],[0 0 1 1],c1);patch([0 1 1 1-e 1-e 0+e],[0 0 1 1-e 0+e 0+e],c2);patch([0 0 1 1-e 0+e 0+e],[0 1 1 1-e 1-e 0+e],c3);plot([0 1 1 0 0],[0 0 1 1 0]);disp('weights');
  "IW{2,1}(687,:)'" : Constant  Value=[0.03640679594455879797276764975322294048964977264404296875;1.41503235135714522385796954040415585041046142578125;-1.34500692658628562270450856885872781276702880859375;-1.4890654429016050297462925300351344048976898193359375;1.0043289558441375053376987125375308096408843994140625;-1.464018689833654018883635217207483947277069091796875;-1.0034899946294186801054593161097727715969085693359375;-1.0280607146917615235537368789664469659328460693359375]
      mask Display: e = 0.06;c1 = [120 150 230]/255;c2 = ([120 150 230]+0)/383;c3 = ([120 150 230]+128)/383;patch([0 1 1 0],[0 0 1 1],c1);patch([0 1 1 1-e 1-e 0+e],[0 0 1 1-e 0+e 0+e],c2);patch([0 0 1 1-e 0+e 0+e],[0 1 1 1-e 1-e 0+e],c3);plot([0 1 1 0 0],[0 0 1 1 0]);disp('weights');
  "IW{2,1}(688,:)'" : Constant  Value=[-1.2450812303516964885119477912667207419872283935546875;0.5143513144949103388370303946430794894695281982421875;-0.85255452959874633567238788600661791861057281494140625;1.6047380508075974603343638591468334197998046875;1.508440339982624056602844575536437332630157470703125;1.16837654486294706401849907706491649150848388671875;1.381438620033878184045761372544802725315093994140625;-0.53344541242854137674811454417067579925060272216796875]
      mask Display: e = 0.06;c1 = [120 150 230]/255;c2 = ([120 150 230]+0)/383;c3 = ([120 150 230]+128)/383;patch([0 1 1 0],[0 0 1 1],c1);patch([0 1 1 1-e 1-e 0+e],[0 0 1 1-e 0+e 0+e],c2);patch([0 0 1 1-e 0+e 0+e],[0 1 1 1-e 1-e 0+e],c3);plot([0 1 1 0 0],[0 0 1 1 0]);disp('weights');
  "IW{2,1}(689,:)'" : Constant  Value=[-1.572546948703477998066091458895243704319000244140625;-1.462176329059851287439641964738257229328155517578125;0.50835714273778809246806531518814153969287872314453125;1.5139796027491196905856440935167483985424041748046875;-0.74158948842218619379451638451428152620792388916015625;0.06385440728651227415557656286182464100420475006103515625;1.107278202194371008459938821033574640750885009765625;-1.4837075338163570048521933131269179284572601318359375]
      mask Display: e = 0.06;c1 = [120 150 230]/255;c2 = ([120 150 230]+0)/383;c3 = ([120 150 230]+128)/383;patch([0 1 1 0],[0 0 1 1],c1);patch([0 1 1 1-e 1-e 0+e],[0 0 1 1-e 0+e 0+e],c2);patch([0 0 1 1-e 0+e 0+e],[0 1 1 1-e 1-e 0+e],c3);plot([0 1 1 0 0],[0 0 1 1 0]);disp('weights');
  "IW{2,1}(69,:)'" : Constant  Value=[-1.5267711745689387381474944049841724336147308349609375;-1.3881718459785175046050653691054321825504302978515625;0.1899210663172064272874450807648827321827411651611328125;-0.37119666898114556108367878550780005753040313720703125;-1.6188613763657586641642183167277835309505462646484375;0.1563589608868909131000890511131728999316692352294921875;-1.67172282734232791057138456380926072597503662109375;-1.16033410230077915770152685581706464290618896484375]
      mask Display: e = 0.06;c1 = [120 150 230]/255;c2 = ([120 150 230]+0)/383;c3 = ([120 150 230]+128)/383;patch([0 1 1 0],[0 0 1 1],c1);patch([0 1 1 1-e 1-e 0+e],[0 0 1 1-e 0+e 0+e],c2);patch([0 0 1 1-e 0+e 0+e],[0 1 1 1-e 1-e 0+e],c3);plot([0 1 1 0 0],[0 0 1 1 0]);disp('weights');
  "IW{2,1}(690,:)'" : Constant  Value=[-0.7052971117884714313817084985203109681606292724609375;1.3476240826866654476390294803422875702381134033203125;-0.5195143804661308539749597912305034697055816650390625;-0.29725318178538751023864961098297499120235443115234375;1.50866845330196053254212529282085597515106201171875;0.7739138245033376772852307112771086394786834716796875;-2.206987021996428044445792693295516073703765869140625;-0.98405920817085446028471551471739076077938079833984375]
      mask Display: e = 0.06;c1 = [120 150 230]/255;c2 = ([120 150 230]+0)/383;c3 = ([120 150 230]+128)/383;patch([0 1 1 0],[0 0 1 1],c1);patch([0 1 1 1-e 1-e 0+e],[0 0 1 1-e 0+e 0+e],c2);patch([0 0 1 1-e 0+e 0+e],[0 1 1 1-e 1-e 0+e],c3);plot([0 1 1 0 0],[0 0 1 1 0]);disp('weights');
  "IW{2,1}(691,:)'" : Constant  Value=[0.56099509856838103427634223407949320971965789794921875;0.06571999828691536815750140476666274480521678924560546875;0.0087796891516778337305471069385021110065281391143798828125;-1.7755031923325379494826847803778946399688720703125;0.421572643564777693736544961211620829999446868896484375;2.521965216402396681161235392210073769092559814453125;0.9804201605191324997434776378213427960872650146484375;-0.328585475275545046969227769295684993267059326171875]
      mask Display: e = 0.06;c1 = [120 150 230]/255;c2 = ([120 150 230]+0)/383;c3 = ([120 150 230]+128)/383;patch([0 1 1 0],[0 0 1 1],c1);patch([0 1 1 1-e 1-e 0+e],[0 0 1 1-e 0+e 0+e],c2);patch([0 0 1 1-e 0+e 0+e],[0 1 1 1-e 1-e 0+e],c3);plot([0 1 1 0 0],[0 0 1 1 0]);disp('weights');
  "IW{2,1}(692,:)'" : Constant  Value=[0.64650173241735486850956249327282421290874481201171875;-0.975201573718762926290537507156841456890106201171875;0.86381755002157201150936316480510868132114410400390625;0.973529448721581314174500221270136535167694091796875;-1.5891568465875345328441881065373308956623077392578125;-1.491734965519403655065389102674089372158050537109375;-0.6627647828545877306538613993325270712375640869140625;1.772364526404005768966953837662003934383392333984375]
      mask Display: e = 0.06;c1 = [120 150 230]/255;c2 = ([120 150 230]+0)/383;c3 = ([120 150 230]+128)/383;patch([0 1 1 0],[0 0 1 1],c1);patch([0 1 1 1-e 1-e 0+e],[0 0 1 1-e 0+e 0+e],c2);patch([0 0 1 1-e 0+e 0+e],[0 1 1 1-e 1-e 0+e],c3);plot([0 1 1 0 0],[0 0 1 1 0]);disp('weights');
  "IW{2,1}(693,:)'" : Constant  Value=[-1.87292279491980284689134350628592073917388916015625;0.60793465062869656012622954222024418413639068603515625;0.10887043302120964771706468354750541038811206817626953125;1.5319889029479536457500898904982022941112518310546875;-1.511305093020176126827891494031064212322235107421875;-0.9681491174858563031335734194726683199405670166015625;0.166628539998758096185582644466194324195384979248046875;1.2202574948246500685655746565316803753376007080078125]
      mask Display: e = 0.06;c1 = [120 150 230]/255;c2 = ([120 150 230]+0)/383;c3 = ([120 150 230]+128)/383;patch([0 1 1 0],[0 0 1 1],c1);patch([0 1 1 1-e 1-e 0+e],[0 0 1 1-e 0+e 0+e],c2);patch([0 0 1 1-e 0+e 0+e],[0 1 1 1-e 1-e 0+e],c3);plot([0 1 1 0 0],[0 0 1 1 0]);disp('weights');
  "IW{2,1}(694,:)'" : Constant  Value=[1.1241482386158787587504548355354927480220794677734375;-1.098229190981534042492739899898879230022430419921875;1.33452742356591347316907558706589043140411376953125;1.8726632019889191127504091127775609493255615234375;0.67994886803567411437398959606071002781391143798828125;-1.3351112588761704369488825250300578773021697998046875;-0.25085050519658802503641936709755100309848785400390625;1.0164843643590140143118105697794817388057708740234375]
      mask Display: e = 0.06;c1 = [120 150 230]/255;c2 = ([120 150 230]+0)/383;c3 = ([120 150 230]+128)/383;patch([0 1 1 0],[0 0 1 1],c1);patch([0 1 1 1-e 1-e 0+e],[0 0 1 1-e 0+e 0+e],c2);patch([0 0 1 1-e 0+e 0+e],[0 1 1 1-e 1-e 0+e],c3);plot([0 1 1 0 0],[0 0 1 1 0]);disp('weights');
  "IW{2,1}(695,:)'" : Constant  Value=[-1.6397319626013306947953651615534909069538116455078125;-1.0612351046851984381902411769260652363300323486328125;-1.619204914366386471868963781162165105342864990234375;-0.2446049206916768581354659772841841913759708404541015625;-0.308738482272347514179244853949057869613170623779296875;1.084514703743274299796439663623459637165069580078125;0.20339414744944706026075209592818282544612884521484375;-1.785943300000659039739048239425756037235260009765625]
      mask Display: e = 0.06;c1 = [120 150 230]/255;c2 = ([120 150 230]+0)/383;c3 = ([120 150 230]+128)/383;patch([0 1 1 0],[0 0 1 1],c1);patch([0 1 1 1-e 1-e 0+e],[0 0 1 1-e 0+e 0+e],c2);patch([0 0 1 1-e 0+e 0+e],[0 1 1 1-e 1-e 0+e],c3);plot([0 1 1 0 0],[0 0 1 1 0]);disp('weights');
  "IW{2,1}(696,:)'" : Constant  Value=[-0.281115725735712584931746960137388668954372406005859375;-1.968149496912217077948525911779142916202545166015625;0.474115775972745401301011725081480108201503753662109375;1.155712134113492606246609284426085650920867919921875;0.13151272963968863027872657767147757112979888916015625;0.813515907622960554590463289059698581695556640625;-1.7802155363690574940704891560017131268978118896484375;-1.284367526319409424928608132177032530307769775390625]
      mask Display: e = 0.06;c1 = [120 150 230]/255;c2 = ([120 150 230]+0)/383;c3 = ([120 150 230]+128)/383;patch([0 1 1 0],[0 0 1 1],c1);patch([0 1 1 1-e 1-e 0+e],[0 0 1 1-e 0+e 0+e],c2);patch([0 0 1 1-e 0+e 0+e],[0 1 1 1-e 1-e 0+e],c3);plot([0 1 1 0 0],[0 0 1 1 0]);disp('weights');
  "IW{2,1}(697,:)'" : Constant  Value=[-1.054956906074191014255347909056581556797027587890625;-1.229017340031933525068552626180462539196014404296875;1.172271732181545456086269041406922042369842529296875;-0.924273388012799568258515137131325900554656982421875;-1.0081071529102747508233051121351309120655059814453125;-1.3634400574116514182065884597250260412693023681640625;1.6034236840494073828011778459767811000347137451171875;0.82034769917917238490900899705593474209308624267578125]
      mask Display: e = 0.06;c1 = [120 150 230]/255;c2 = ([120 150 230]+0)/383;c3 = ([120 150 230]+128)/383;patch([0 1 1 0],[0 0 1 1],c1);patch([0 1 1 1-e 1-e 0+e],[0 0 1 1-e 0+e 0+e],c2);patch([0 0 1 1-e 0+e 0+e],[0 1 1 1-e 1-e 0+e],c3);plot([0 1 1 0 0],[0 0 1 1 0]);disp('weights');
  "IW{2,1}(698,:)'" : Constant  Value=[-0.1651064052522357439301003978471271693706512451171875;1.743618673268698682221611306886188685894012451171875;-0.0462034908411141087558604567675502039492130279541015625;-0.8313589700909786994742489696363918483257293701171875;-0.1927763030832403412517805918469093739986419677734375;2.028223001746049636295765594695694744586944580078125;0.33819199573463476493628832031390629708766937255859375;1.7016002348315300007897121759015135467052459716796875]
      mask Display: e = 0.06;c1 = [120 150 230]/255;c2 = ([120 150 230]+0)/383;c3 = ([120 150 230]+128)/383;patch([0 1 1 0],[0 0 1 1],c1);patch([0 1 1 1-e 1-e 0+e],[0 0 1 1-e 0+e 0+e],c2);patch([0 0 1 1-e 0+e 0+e],[0 1 1 1-e 1-e 0+e],c3);plot([0 1 1 0 0],[0 0 1 1 0]);disp('weights');
  "IW{2,1}(699,:)'" : Constant  Value=[0.882770970531875587283821005257777869701385498046875;0.09423724212022772939167936101512168534100055694580078125;0.87819834418356002014860450799460522830486297607421875;0.73704703660963588607302199307014234364032745361328125;-1.495233672388470491654288707650266587734222412109375;-1.6945873118049326055967185311601497232913970947265625;-1.9567504008844489593599291765713132917881011962890625;0.07744293702652259303587101157972938381135463714599609375]
      mask Display: e = 0.06;c1 = [120 150 230]/255;c2 = ([120 150 230]+0)/383;c3 = ([120 150 230]+128)/383;patch([0 1 1 0],[0 0 1 1],c1);patch([0 1 1 1-e 1-e 0+e],[0 0 1 1-e 0+e 0+e],c2);patch([0 0 1 1-e 0+e 0+e],[0 1 1 1-e 1-e 0+e],c3);plot([0 1 1 0 0],[0 0 1 1 0]);disp('weights');
  "IW{2,1}(7,:)'" : Constant  Value=[0.5012126299523789185741406981833279132843017578125;-1.265361209579563439575622396660037338733673095703125;1.3300380397611253346923376739141531288623809814453125;1.2515642450334656388122311909683048725128173828125;-1.306290581060304933913585045957006514072418212890625;-1.187047720391800620376443475834093987941741943359375;1.2516661317004935671803877994534559547901153564453125;1.035248957783328815906997988349758088588714599609375]
      mask Display: e = 0.06;c1 = [120 150 230]/255;c2 = ([120 150 230]+0)/383;c3 = ([120 150 230]+128)/383;patch([0 1 1 0],[0 0 1 1],c1);patch([0 1 1 1-e 1-e 0+e],[0 0 1 1-e 0+e 0+e],c2);patch([0 0 1 1-e 0+e 0+e],[0 1 1 1-e 1-e 0+e],c3);plot([0 1 1 0 0],[0 0 1 1 0]);disp('weights');
  "IW{2,1}(70,:)'" : Constant  Value=[1.97055540507814175299472481128759682178497314453125;-0.54828781919186087012718644473352469503879547119140625;-1.1950866320718713797788268493604846298694610595703125;-0.938835840301493362858309410512447357177734375;2.00996025538912537200531005510129034519195556640625;0.297304169484826241731667550993734039366245269775390625;-0.691492114820844161471313782385550439357757568359375;-0.27731097289654293991389977236394770443439483642578125]
      mask Display: e = 0.06;c1 = [120 150 230]/255;c2 = ([120 150 230]+0)/383;c3 = ([120 150 230]+128)/383;patch([0 1 1 0],[0 0 1 1],c1);patch([0 1 1 1-e 1-e 0+e],[0 0 1 1-e 0+e 0+e],c2);patch([0 0 1 1-e 0+e 0+e],[0 1 1 1-e 1-e 0+e],c3);plot([0 1 1 0 0],[0 0 1 1 0]);disp('weights');
  "IW{2,1}(700,:)'" : Constant  Value=[-1.801281605187828205316691310144960880279541015625;-0.48420103168596029252768175865639932453632354736328125;-0.465996379431057261566451188627979718148708343505859375;1.727449140805457528102806463721208274364471435546875;-0.60058222319921006349119352307752706110477447509765625;-1.3930969671030251078036599210463464260101318359375;1.34803717318590177143278197036124765872955322265625;-0.424713718591940903035464316417346708476543426513671875]
      mask Display: e = 0.06;c1 = [120 150 230]/255;c2 = ([120 150 230]+0)/383;c3 = ([120 150 230]+128)/383;patch([0 1 1 0],[0 0 1 1],c1);patch([0 1 1 1-e 1-e 0+e],[0 0 1 1-e 0+e 0+e],c2);patch([0 0 1 1-e 0+e 0+e],[0 1 1 1-e 1-e 0+e],c3);plot([0 1 1 0 0],[0 0 1 1 0]);disp('weights');
  "IW{2,1}(701,:)'" : Constant  Value=[1.017071030056532432439553303993307054042816162109375;-0.55378002550578886431509317844756878912448883056640625;1.0516780081951744296731021677260287106037139892578125;0.231523049605480479851138397862087003886699676513671875;-2.15797481608037511335851377225480973720550537109375;-0.8180620885015315035815319788525812327861785888671875;-1.0794061375938335256563505026861093938350677490234375;1.4639881543919919248963878999347798526287078857421875]
      mask Display: e = 0.06;c1 = [120 150 230]/255;c2 = ([120 150 230]+0)/383;c3 = ([120 150 230]+128)/383;patch([0 1 1 0],[0 0 1 1],c1);patch([0 1 1 1-e 1-e 0+e],[0 0 1 1-e 0+e 0+e],c2);patch([0 0 1 1-e 0+e 0+e],[0 1 1 1-e 1-e 0+e],c3);plot([0 1 1 0 0],[0 0 1 1 0]);disp('weights');
  "IW{2,1}(702,:)'" : Constant  Value=[1.808230400030936824151694963802583515644073486328125;0.705584950502672558769745592144317924976348876953125;-0.64276880643120082314823093838640488684177398681640625;-0.6761449622810669080053003199282102286815643310546875;-2.03962247967967158501778612844645977020263671875;-0.8381190445033082081494058002135716378688812255859375;1.178584707401815645511078400886617600917816162109375;0.32793678103610801599643309600651264190673828125]
      mask Display: e = 0.06;c1 = [120 150 230]/255;c2 = ([120 150 230]+0)/383;c3 = ([120 150 230]+128)/383;patch([0 1 1 0],[0 0 1 1],c1);patch([0 1 1 1-e 1-e 0+e],[0 0 1 1-e 0+e 0+e],c2);patch([0 0 1 1-e 0+e 0+e],[0 1 1 1-e 1-e 0+e],c3);plot([0 1 1 0 0],[0 0 1 1 0]);disp('weights');
  "IW{2,1}(703,:)'" : Constant  Value=[-1.974985011322868633243388103437609970569610595703125;-1.574587469006125228787595915491692721843719482421875;-0.21839437443907794289543744525872170925140380859375;-1.1144203892674358069569962026434950530529022216796875;-0.61941059932116038222460474571562372148036956787109375;-0.292888388722526149532399131203419528901576995849609375;0.5158141346634235180346195193124003708362579345703125;1.608168693488261080659640356316231191158294677734375]
      mask Display: e = 0.06;c1 = [120 150 230]/255;c2 = ([120 150 230]+0)/383;c3 = ([120 150 230]+128)/383;patch([0 1 1 0],[0 0 1 1],c1);patch([0 1 1 1-e 1-e 0+e],[0 0 1 1-e 0+e 0+e],c2);patch([0 0 1 1-e 0+e 0+e],[0 1 1 1-e 1-e 0+e],c3);plot([0 1 1 0 0],[0 0 1 1 0]);disp('weights');
  "IW{2,1}(704,:)'" : Constant  Value=[0.069047459673273248181857297822716645896434783935546875;0.336472797214267760335104640034842304885387420654296875;-0.4599753479369315112279537061112932860851287841796875;-0.5043848918265754210921159028657712042331695556640625;-1.8420934501433603447395626062643714249134063720703125;2.222078583025664411110255969106219708919525146484375;0.1907136794964536807839294851874001324176788330078125;1.44624677017538960654974289354868233203887939453125]
      mask Display: e = 0.06;c1 = [120 150 230]/255;c2 = ([120 150 230]+0)/383;c3 = ([120 150 230]+128)/383;patch([0 1 1 0],[0 0 1 1],c1);patch([0 1 1 1-e 1-e 0+e],[0 0 1 1-e 0+e 0+e],c2);patch([0 0 1 1-e 0+e 0+e],[0 1 1 1-e 1-e 0+e],c3);plot([0 1 1 0 0],[0 0 1 1 0]);disp('weights');
  "IW{2,1}(705,:)'" : Constant  Value=[2.04707548105371817115383237251080572605133056640625;-1.3096051615007182622463233201415278017520904541015625;-2.18851473967893372929438555729575455188751220703125;0.1919441891947284151154207165745901875197887420654296875;-0.24287695201083725482504860337940044701099395751953125;0.320089093041101169223594524737563915550708770751953125;0.1471570486326387039444085758077562786638736724853515625;-0.1570113383726058076117482187328278087079524993896484375]
      mask Display: e = 0.06;c1 = [120 150 230]/255;c2 = ([120 150 230]+0)/383;c3 = ([120 150 230]+128)/383;patch([0 1 1 0],[0 0 1 1],c1);patch([0 1 1 1-e 1-e 0+e],[0 0 1 1-e 0+e 0+e],c2);patch([0 0 1 1-e 0+e 0+e],[0 1 1 1-e 1-e 0+e],c3);plot([0 1 1 0 0],[0 0 1 1 0]);disp('weights');
  "IW{2,1}(706,:)'" : Constant  Value=[-1.147798347369108018511951740947552025318145751953125;-0.629707611259006316828390481532551348209381103515625;-0.294844763829132328059046130874776281416416168212890625;1.1430543183962498243744221326778642833232879638671875;2.112555822708354735794955558958463370800018310546875;0.126132620440300768915875551101635210216045379638671875;-1.8369410457691477400743451653397642076015472412109375;-0.264066481740402370093079298385418951511383056640625]
      mask Display: e = 0.06;c1 = [120 150 230]/255;c2 = ([120 150 230]+0)/383;c3 = ([120 150 230]+128)/383;patch([0 1 1 0],[0 0 1 1],c1);patch([0 1 1 1-e 1-e 0+e],[0 0 1 1-e 0+e 0+e],c2);patch([0 0 1 1-e 0+e 0+e],[0 1 1 1-e 1-e 0+e],c3);plot([0 1 1 0 0],[0 0 1 1 0]);disp('weights');
  "IW{2,1}(707,:)'" : Constant  Value=[1.0391415186058206021613159464322961866855621337890625;2.0660867250717824816774736973457038402557373046875;-0.6133529936427246642693944522761739790439605712890625;0.73177641089810385732761233157361857593059539794921875;1.3603453439010924075347475081798620522022247314453125;-0.38899408109859745508174455608241260051727294921875;1.443594287652115060183177774888463318347930908203125;0.80776414067460089452055171932443045079708099365234375]
      mask Display: e = 0.06;c1 = [120 150 230]/255;c2 = ([120 150 230]+0)/383;c3 = ([120 150 230]+128)/383;patch([0 1 1 0],[0 0 1 1],c1);patch([0 1 1 1-e 1-e 0+e],[0 0 1 1-e 0+e 0+e],c2);patch([0 0 1 1-e 0+e 0+e],[0 1 1 1-e 1-e 0+e],c3);plot([0 1 1 0 0],[0 0 1 1 0]);disp('weights');
  "IW{2,1}(708,:)'" : Constant  Value=[-1.0507806121373388652529001774382777512073516845703125;-0.95169224119408368789407859367202036082744598388671875;1.0382028536618246317146940782549791038036346435546875;-1.4323748251546180032534039128222502768039703369140625;-1.6735107304301346520247761873179115355014801025390625;-1.3772611359687882970348482558620162308216094970703125;-1.01363131979757259415464432095177471637725830078125;-0.36767019529963873569755605785758234560489654541015625]
      mask Display: e = 0.06;c1 = [120 150 230]/255;c2 = ([120 150 230]+0)/383;c3 = ([120 150 230]+128)/383;patch([0 1 1 0],[0 0 1 1],c1);patch([0 1 1 1-e 1-e 0+e],[0 0 1 1-e 0+e 0+e],c2);patch([0 0 1 1-e 0+e 0+e],[0 1 1 1-e 1-e 0+e],c3);plot([0 1 1 0 0],[0 0 1 1 0]);disp('weights');
  "IW{2,1}(709,:)'" : Constant  Value=[-0.422340079736405360488760152293252758681774139404296875;0.9065676361928705073722767338040284812450408935546875;-0.75941237075621648155987486461526714265346527099609375;1.53572131965478941850733463070355355739593505859375;-1.44851190435536647527214881847612559795379638671875;-1.794907788810011783908748839166946709156036376953125;0.9753309032726160676673998750629834830760955810546875;-0.9076680058968340514269357299781404435634613037109375]
      mask Display: e = 0.06;c1 = [120 150 230]/255;c2 = ([120 150 230]+0)/383;c3 = ([120 150 230]+128)/383;patch([0 1 1 0],[0 0 1 1],c1);patch([0 1 1 1-e 1-e 0+e],[0 0 1 1-e 0+e 0+e],c2);patch([0 0 1 1-e 0+e 0+e],[0 1 1 1-e 1-e 0+e],c3);plot([0 1 1 0 0],[0 0 1 1 0]);disp('weights');
  "IW{2,1}(71,:)'" : Constant  Value=[-2.197401939083988953171910907258279621601104736328125;0.322868715528588812180288414310780353844165802001953125;1.47813042897090429761419727583415806293487548828125;-0.5767621887840734817842758275219239294528961181640625;-0.73765800656971503013181745700421743094921112060546875;-0.65279531279554914302565293837687931954860687255859375;-0.44557911148788653665775427725748158991336822509765625;-1.4078284004324161937660164767294190824031829833984375]
      mask Display: e = 0.06;c1 = [120 150 230]/255;c2 = ([120 150 230]+0)/383;c3 = ([120 150 230]+128)/383;patch([0 1 1 0],[0 0 1 1],c1);patch([0 1 1 1-e 1-e 0+e],[0 0 1 1-e 0+e 0+e],c2);patch([0 0 1 1-e 0+e 0+e],[0 1 1 1-e 1-e 0+e],c3);plot([0 1 1 0 0],[0 0 1 1 0]);disp('weights');
  "IW{2,1}(710,:)'" : Constant  Value=[-1.236950703614706714716930946451611816883087158203125;-0.12987822000432280855619637804920785129070281982421875;-0.85395230872580896175350062549114227294921875;0.810266929743658881335477417451329529285430908203125;-1.2560468896706276087371634275768883526325225830078125;-0.30407637893327488232131372569710947573184967041015625;-0.0635349245639229565085770445875823497772216796875;-2.529097404542338001220969090354628860950469970703125]
      mask Display: e = 0.06;c1 = [120 150 230]/255;c2 = ([120 150 230]+0)/383;c3 = ([120 150 230]+128)/383;patch([0 1 1 0],[0 0 1 1],c1);patch([0 1 1 1-e 1-e 0+e],[0 0 1 1-e 0+e 0+e],c2);patch([0 0 1 1-e 0+e 0+e],[0 1 1 1-e 1-e 0+e],c3);plot([0 1 1 0 0],[0 0 1 1 0]);disp('weights');
  "IW{2,1}(711,:)'" : Constant  Value=[-0.022636762249209664565885447018445120193064212799072265625;-1.4117876203082999619908832755754701793193817138671875;-0.0100619509587923823545896340192484785802662372589111328125;1.6579100689682573221972461396944709122180938720703125;0.48474053427652241676781841306365095078945159912109375;1.5540990148452185071192843679455108940601348876953125;-0.367818936142799757238464053443749435245990753173828125;1.8530609953077477047855836644885130226612091064453125]
      mask Display: e = 0.06;c1 = [120 150 230]/255;c2 = ([120 150 230]+0)/383;c3 = ([120 150 230]+128)/383;patch([0 1 1 0],[0 0 1 1],c1);patch([0 1 1 1-e 1-e 0+e],[0 0 1 1-e 0+e 0+e],c2);patch([0 0 1 1-e 0+e 0+e],[0 1 1 1-e 1-e 0+e],c3);plot([0 1 1 0 0],[0 0 1 1 0]);disp('weights');
  "IW{2,1}(712,:)'" : Constant  Value=[1.5341347884280944757762199515127576887607574462890625;0.315588272669764802191849639712017960846424102783203125;-1.5597337307381831106312120027723722159862518310546875;-1.5666493829117740244072365385363809764385223388671875;-1.33623144467710286420469856238923966884613037109375;0.384590608874562589480916585671366192400455474853515625;0.09155979535125786938909442369549651630222797393798828125;-1.320630447580561028786405586288310587406158447265625]
      mask Display: e = 0.06;c1 = [120 150 230]/255;c2 = ([120 150 230]+0)/383;c3 = ([120 150 230]+128)/383;patch([0 1 1 0],[0 0 1 1],c1);patch([0 1 1 1-e 1-e 0+e],[0 0 1 1-e 0+e 0+e],c2);patch([0 0 1 1-e 0+e 0+e],[0 1 1 1-e 1-e 0+e],c3);plot([0 1 1 0 0],[0 0 1 1 0]);disp('weights');
  "IW{2,1}(713,:)'" : Constant  Value=[-0.44932803724355496743925186819978989660739898681640625;-0.38568941562783010112980264239013195037841796875;-1.3658559779548660184644859327818267047405242919921875;1.730911973146498805675719268037937581539154052734375;-0.87551876366416447883267437646281905472278594970703125;-2.218690641127498253126759664155542850494384765625;-0.1437719267851877702479868048612843267619609832763671875;0.2830538740401653541312043671496212482452392578125]
      mask Display: e = 0.06;c1 = [120 150 230]/255;c2 = ([120 150 230]+0)/383;c3 = ([120 150 230]+128)/383;patch([0 1 1 0],[0 0 1 1],c1);patch([0 1 1 1-e 1-e 0+e],[0 0 1 1-e 0+e 0+e],c2);patch([0 0 1 1-e 0+e 0+e],[0 1 1 1-e 1-e 0+e],c3);plot([0 1 1 0 0],[0 0 1 1 0]);disp('weights');
  "IW{2,1}(714,:)'" : Constant  Value=[0.1205014965027775553085831461430643685162067413330078125;-1.710076262052667939173034028499387204647064208984375;0.87780001710598132280694017026689834892749786376953125;-1.3354744101665136923884347197599709033966064453125;0.50281356389044429278101233649067580699920654296875;2.045958651236494230118978521204553544521331787109375;0.92724312876308301323291516382596455514430999755859375;-0.451615397991576961178594729062751866877079010009765625]
      mask Display: e = 0.06;c1 = [120 150 230]/255;c2 = ([120 150 230]+0)/383;c3 = ([120 150 230]+128)/383;patch([0 1 1 0],[0 0 1 1],c1);patch([0 1 1 1-e 1-e 0+e],[0 0 1 1-e 0+e 0+e],c2);patch([0 0 1 1-e 0+e 0+e],[0 1 1 1-e 1-e 0+e],c3);plot([0 1 1 0 0],[0 0 1 1 0]);disp('weights');
  "IW{2,1}(715,:)'" : Constant  Value=[0.1384014317495194656970625146641395986080169677734375;1.6961884232562420837808758733444847166538238525390625;-1.2097574264073234218130892259068787097930908203125;2.0493567213227361634153567138127982616424560546875;-0.6741290006757407748949617598555050790309906005859375;-0.00909531327803718425695223004368017427623271942138671875;-1.104194540942956326290413926471956074237823486328125;-0.93215582126154294950737266844953410327434539794921875]
      mask Display: e = 0.06;c1 = [120 150 230]/255;c2 = ([120 150 230]+0)/383;c3 = ([120 150 230]+128)/383;patch([0 1 1 0],[0 0 1 1],c1);patch([0 1 1 1-e 1-e 0+e],[0 0 1 1-e 0+e 0+e],c2);patch([0 0 1 1-e 0+e 0+e],[0 1 1 1-e 1-e 0+e],c3);plot([0 1 1 0 0],[0 0 1 1 0]);disp('weights');
  "IW{2,1}(716,:)'" : Constant  Value=[-1.59726558824709830020083245472051203250885009765625;1.76645162714476899878945914679206907749176025390625;0.231488386123363198976221610791981220245361328125;-0.475241444399484291860602525048307143151760101318359375;1.065095764085777663154885885887779295444488525390625;-0.478198194603901283183944315169355832040309906005859375;-1.62102513511541257429371398757211863994598388671875;-1.0208323375184662484826958461781032383441925048828125]
      mask Display: e = 0.06;c1 = [120 150 230]/255;c2 = ([120 150 230]+0)/383;c3 = ([120 150 230]+128)/383;patch([0 1 1 0],[0 0 1 1],c1);patch([0 1 1 1-e 1-e 0+e],[0 0 1 1-e 0+e 0+e],c2);patch([0 0 1 1-e 0+e 0+e],[0 1 1 1-e 1-e 0+e],c3);plot([0 1 1 0 0],[0 0 1 1 0]);disp('weights');
  "IW{2,1}(717,:)'" : Constant  Value=[-0.99759930109675465370600022652070038020610809326171875;-0.86534818743351282765985388323315419256687164306640625;-0.495069912277181278792426155632711015641689300537109375;-0.06545907481878800171504195759553113020956516265869140625;2.07600632899209980308796730241738259792327880859375;-0.280082667658566986101931206576409749686717987060546875;1.101114597942876027758529744460247457027435302734375;-1.9217321098241828547514842284726910293102264404296875]
      mask Display: e = 0.06;c1 = [120 150 230]/255;c2 = ([120 150 230]+0)/383;c3 = ([120 150 230]+128)/383;patch([0 1 1 0],[0 0 1 1],c1);patch([0 1 1 1-e 1-e 0+e],[0 0 1 1-e 0+e 0+e],c2);patch([0 0 1 1-e 0+e 0+e],[0 1 1 1-e 1-e 0+e],c3);plot([0 1 1 0 0],[0 0 1 1 0]);disp('weights');
  "IW{2,1}(718,:)'" : Constant  Value=[-0.62213697436987802635854905020096339285373687744140625;1.82911295499014414644989301450550556182861328125;0.92571391648267009610862032786826603114604949951171875;-1.7265979309417744946841821729321964085102081298828125;0.310747453372343496180718602772685699164867401123046875;-1.18178242373057695857596627320162951946258544921875;-0.035173179724109375487994810782765853218734264373779296875;-1.501866228599948893673854399821721017360687255859375]
      mask Display: e = 0.06;c1 = [120 150 230]/255;c2 = ([120 150 230]+0)/383;c3 = ([120 150 230]+128)/383;patch([0 1 1 0],[0 0 1 1],c1);patch([0 1 1 1-e 1-e 0+e],[0 0 1 1-e 0+e 0+e],c2);patch([0 0 1 1-e 0+e 0+e],[0 1 1 1-e 1-e 0+e],c3);plot([0 1 1 0 0],[0 0 1 1 0]);disp('weights');
  "IW{2,1}(719,:)'" : Constant  Value=[-2.085239574961076147729954755050130188465118408203125;0.1698165194862840954304061824586824513971805572509765625;0.621367472909037932282672045403160154819488525390625;-1.9351364415996872292424768602359108626842498779296875;1.209649864605828017971589360968209803104400634765625;0.468363831993300727685181072956766001880168914794921875;0.69078422426405483580680311206378974020481109619140625;-0.0797827617237958641727146869015996344387531280517578125]
      mask Display: e = 0.06;c1 = [120 150 230]/255;c2 = ([120 150 230]+0)/383;c3 = ([120 150 230]+128)/383;patch([0 1 1 0],[0 0 1 1],c1);patch([0 1 1 1-e 1-e 0+e],[0 0 1 1-e 0+e 0+e],c2);patch([0 0 1 1-e 0+e 0+e],[0 1 1 1-e 1-e 0+e],c3);plot([0 1 1 0 0],[0 0 1 1 0]);disp('weights');
  "IW{2,1}(72,:)'" : Constant  Value=[-1.7272272479745964801622903905808925628662109375;-0.722643755597194736850497065461240708827972412109375;-0.678424234205483589477125860867090523242950439453125;-0.72574730192308389842281712844851426780223846435546875;1.052143387268287266778088451246730983257293701171875;-1.765348684504318033106073926319368183612823486328125;1.4743780797510179780829275841824710369110107421875;0.61802781886638558095370399314560927450656890869140625]
      mask Display: e = 0.06;c1 = [120 150 230]/255;c2 = ([120 150 230]+0)/383;c3 = ([120 150 230]+128)/383;patch([0 1 1 0],[0 0 1 1],c1);patch([0 1 1 1-e 1-e 0+e],[0 0 1 1-e 0+e 0+e],c2);patch([0 0 1 1-e 0+e 0+e],[0 1 1 1-e 1-e 0+e],c3);plot([0 1 1 0 0],[0 0 1 1 0]);disp('weights');
  "IW{2,1}(720,:)'" : Constant  Value=[-1.010718354928799467273847767501138150691986083984375;1.2303541999668630158026871868059970438480377197265625;1.6785296275035179736079271606286056339740753173828125;1.2385554601692521092815013616927899420261383056640625;-0.94475503232582236368131134440773166716098785400390625;0.808107171012599767578876708284951746463775634765625;-0.45337771114326053112364434127812273800373077392578125;-1.512422119707868883864421150065027177333831787109375]
      mask Display: e = 0.06;c1 = [120 150 230]/255;c2 = ([120 150 230]+0)/383;c3 = ([120 150 230]+128)/383;patch([0 1 1 0],[0 0 1 1],c1);patch([0 1 1 1-e 1-e 0+e],[0 0 1 1-e 0+e 0+e],c2);patch([0 0 1 1-e 0+e 0+e],[0 1 1 1-e 1-e 0+e],c3);plot([0 1 1 0 0],[0 0 1 1 0]);disp('weights');
  "IW{2,1}(721,:)'" : Constant  Value=[1.2454680165485425558102861032239161431789398193359375;0.35793180515564582133691828857990913093090057373046875;-0.27439006305087010328946917070425115525722503662109375;1.4239821714230382898591642515384592115879058837890625;-0.467863986816844434901696558881667442619800567626953125;-1.0730683775352460873619975245674140751361846923828125;-1.1764765497179745512568160847877152264118194580078125;-2.16612562126943064555462115094996988773345947265625]
      mask Display: e = 0.06;c1 = [120 150 230]/255;c2 = ([120 150 230]+0)/383;c3 = ([120 150 230]+128)/383;patch([0 1 1 0],[0 0 1 1],c1);patch([0 1 1 1-e 1-e 0+e],[0 0 1 1-e 0+e 0+e],c2);patch([0 0 1 1-e 0+e 0+e],[0 1 1 1-e 1-e 0+e],c3);plot([0 1 1 0 0],[0 0 1 1 0]);disp('weights');
  "IW{2,1}(722,:)'" : Constant  Value=[1.6195523113503396128720623892149887979030609130859375;0.0372680507794286575151687657125876285135746002197265625;0.71717148287294973929562047487706877291202545166015625;-0.277972858935977951144735698107979260385036468505859375;0.422413596248763456575403552051284350454807281494140625;-1.9730307927564629810746055227355100214481353759765625;-0.68038021296147455085900901394779793918132781982421875;-1.8627128554503975532696813388611190021038055419921875]
      mask Display: e = 0.06;c1 = [120 150 230]/255;c2 = ([120 150 230]+0)/383;c3 = ([120 150 230]+128)/383;patch([0 1 1 0],[0 0 1 1],c1);patch([0 1 1 1-e 1-e 0+e],[0 0 1 1-e 0+e 0+e],c2);patch([0 0 1 1-e 0+e 0+e],[0 1 1 1-e 1-e 0+e],c3);plot([0 1 1 0 0],[0 0 1 1 0]);disp('weights');
  "IW{2,1}(723,:)'" : Constant  Value=[0.9938895596005730137534328605397604405879974365234375;0.62284114637445442408392182187526486814022064208984375;-1.89298694396008659879271363024599850177764892578125;-0.316464325822178038638554653516621328890323638916015625;-0.7538345961142838280721889532287605106830596923828125;-0.75404152458469619890735202716314233839511871337890625;-0.8264748095158316321118263658718205988407135009765625;-2.082829913662715970446015489869751036167144775390625]
      mask Display: e = 0.06;c1 = [120 150 230]/255;c2 = ([120 150 230]+0)/383;c3 = ([120 150 230]+128)/383;patch([0 1 1 0],[0 0 1 1],c1);patch([0 1 1 1-e 1-e 0+e],[0 0 1 1-e 0+e 0+e],c2);patch([0 0 1 1-e 0+e 0+e],[0 1 1 1-e 1-e 0+e],c3);plot([0 1 1 0 0],[0 0 1 1 0]);disp('weights');
  "IW{2,1}(724,:)'" : Constant  Value=[-1.79172106030249711494661823962815105915069580078125;-1.4087218708695277147313618115731514990329742431640625;0.88197075391598733773435014882124960422515869140625;-0.06598171940630508103264872943327645771205425262451171875;-0.197143566113255730432030077281524427235126495361328125;-2.11355389131774895616899812011979520320892333984375;0.689704751178218611329384657437913119792938232421875;0.323772462258188176154050097466097213327884674072265625]
      mask Display: e = 0.06;c1 = [120 150 230]/255;c2 = ([120 150 230]+0)/383;c3 = ([120 150 230]+128)/383;patch([0 1 1 0],[0 0 1 1],c1);patch([0 1 1 1-e 1-e 0+e],[0 0 1 1-e 0+e 0+e],c2);patch([0 0 1 1-e 0+e 0+e],[0 1 1 1-e 1-e 0+e],c3);plot([0 1 1 0 0],[0 0 1 1 0]);disp('weights');
  "IW{2,1}(725,:)'" : Constant  Value=[-0.94250755904706551291383220814168453216552734375;1.79629372061520431458347957232035696506500244140625;0.722821793370013399027129707974381744861602783203125;0.097860467375111337418047696701250970363616943359375;-1.6513816787943518260561859278823249042034149169921875;1.7412624095466771034779185356455855071544647216796875;-0.0710882652791876290532258053644909523427486419677734375;0.733109503109491189576374381431378424167633056640625]
      mask Display: e = 0.06;c1 = [120 150 230]/255;c2 = ([120 150 230]+0)/383;c3 = ([120 150 230]+128)/383;patch([0 1 1 0],[0 0 1 1],c1);patch([0 1 1 1-e 1-e 0+e],[0 0 1 1-e 0+e 0+e],c2);patch([0 0 1 1-e 0+e 0+e],[0 1 1 1-e 1-e 0+e],c3);plot([0 1 1 0 0],[0 0 1 1 0]);disp('weights');
  "IW{2,1}(726,:)'" : Constant  Value=[-0.9294554917103992064397743888548575341701507568359375;1.6747228465754384618691119612776674330234527587890625;-0.492437814456765876602872822331846691668033599853515625;-1.475015803112942336383639485575258731842041015625;1.649136414041774134631168635678477585315704345703125;1.1214370607177726046899124412448145449161529541015625;0.75586758900522166282343050625058822333812713623046875;-0.5310018450362734565572964129387401044368743896484375]
      mask Display: e = 0.06;c1 = [120 150 230]/255;c2 = ([120 150 230]+0)/383;c3 = ([120 150 230]+128)/383;patch([0 1 1 0],[0 0 1 1],c1);patch([0 1 1 1-e 1-e 0+e],[0 0 1 1-e 0+e 0+e],c2);patch([0 0 1 1-e 0+e 0+e],[0 1 1 1-e 1-e 0+e],c3);plot([0 1 1 0 0],[0 0 1 1 0]);disp('weights');
  "IW{2,1}(727,:)'" : Constant  Value=[-0.2022739756581155290415807712633977644145488739013671875;1.68326488021440123787897391594015061855316162109375;-0.438219939296272842366164468330680392682552337646484375;0.990526156885977560051514956285245716571807861328125;-0.271973287136569263910956806284957565367221832275390625;1.6489262835942495311059019513777457177639007568359375;-0.4529319581668034278010281923343427479267120361328125;-1.96725077933217296077827995759434998035430908203125]
      mask Display: e = 0.06;c1 = [120 150 230]/255;c2 = ([120 150 230]+0)/383;c3 = ([120 150 230]+128)/383;patch([0 1 1 0],[0 0 1 1],c1);patch([0 1 1 1-e 1-e 0+e],[0 0 1 1-e 0+e 0+e],c2);patch([0 0 1 1-e 0+e 0+e],[0 1 1 1-e 1-e 0+e],c3);plot([0 1 1 0 0],[0 0 1 1 0]);disp('weights');
  "IW{2,1}(728,:)'" : Constant  Value=[0.369864007182385712280137113339151255786418914794921875;1.8053906967409110162492424933589063584804534912109375;-1.82050878346358846471275683143176138401031494140625;-1.4971838796865604148678130513872019946575164794921875;0.11394603858829925602247357119267689995467662811279296875;-0.6323478480591926409459802016499452292919158935546875;0.98879482885230507438478753101662732660770416259765625;0.831161490443918182791094295680522918701171875]
      mask Display: e = 0.06;c1 = [120 150 230]/255;c2 = ([120 150 230]+0)/383;c3 = ([120 150 230]+128)/383;patch([0 1 1 0],[0 0 1 1],c1);patch([0 1 1 1-e 1-e 0+e],[0 0 1 1-e 0+e 0+e],c2);patch([0 0 1 1-e 0+e 0+e],[0 1 1 1-e 1-e 0+e],c3);plot([0 1 1 0 0],[0 0 1 1 0]);disp('weights');
  "IW{2,1}(729,:)'" : Constant  Value=[0.554310451896775635560743467067368328571319580078125;-1.536431058643708436051156240864656865596771240234375;1.8006025158723020229700750860502012073993682861328125;1.7099450794714765589077387630823068320751190185546875;-1.3732289607365639749758656762423925101757049560546875;0.59363643914777741716903847191133536398410797119140625;0.0753611809343303906683075865657883696258068084716796875;-0.2240793845090387204077586602579685859382152557373046875]
      mask Display: e = 0.06;c1 = [120 150 230]/255;c2 = ([120 150 230]+0)/383;c3 = ([120 150 230]+128)/383;patch([0 1 1 0],[0 0 1 1],c1);patch([0 1 1 1-e 1-e 0+e],[0 0 1 1-e 0+e 0+e],c2);patch([0 0 1 1-e 0+e 0+e],[0 1 1 1-e 1-e 0+e],c3);plot([0 1 1 0 0],[0 0 1 1 0]);disp('weights');
  "IW{2,1}(73,:)'" : Constant  Value=[0.55873224076399286008864919494953937828540802001953125;0.143965331046209621401743561364128254354000091552734375;1.348270961588249772233893963857553899288177490234375;1.3286142568428207511033178889192640781402587890625;-0.197143599737428842910702542212675325572490692138671875;2.332618171148955976690331226564012467861175537109375;0.179649882950733863484771291041397489607334136962890625;-1.3399169631518865752894953402574174106121063232421875]
      mask Display: e = 0.06;c1 = [120 150 230]/255;c2 = ([120 150 230]+0)/383;c3 = ([120 150 230]+128)/383;patch([0 1 1 0],[0 0 1 1],c1);patch([0 1 1 1-e 1-e 0+e],[0 0 1 1-e 0+e 0+e],c2);patch([0 0 1 1-e 0+e 0+e],[0 1 1 1-e 1-e 0+e],c3);plot([0 1 1 0 0],[0 0 1 1 0]);disp('weights');
  "IW{2,1}(730,:)'" : Constant  Value=[-1.075735991095414068041691280086524784564971923828125;1.9114745754246598163916814883123151957988739013671875;-0.26326360278689531213558439048938453197479248046875;-1.7716140222876231025139759367448277771472930908203125;0.98842314725460855839855867088772356510162353515625;0.09552333282607218534199233772596926428377628326416015625;0.3126453510906455068862896951031871140003204345703125;-1.4725866055501961593421356155886314809322357177734375]
      mask Display: e = 0.06;c1 = [120 150 230]/255;c2 = ([120 150 230]+0)/383;c3 = ([120 150 230]+128)/383;patch([0 1 1 0],[0 0 1 1],c1);patch([0 1 1 1-e 1-e 0+e],[0 0 1 1-e 0+e 0+e],c2);patch([0 0 1 1-e 0+e 0+e],[0 1 1 1-e 1-e 0+e],c3);plot([0 1 1 0 0],[0 0 1 1 0]);disp('weights');
  "IW{2,1}(731,:)'" : Constant  Value=[-1.4050294766007291880072216372354887425899505615234375;-0.98112127095895040884698801164631731808185577392578125;1.5718622011789127324021819731569848954677581787109375;-1.1230412074393267829464093665592372417449951171875;-1.82390204833623581492929588421247899532318115234375;-0.006662581433525704803499944972600133041851222515106201171875;0.9809684139897487664683239927398972213268280029296875;0.24775192630758724465778186640818603336811065673828125]
      mask Display: e = 0.06;c1 = [120 150 230]/255;c2 = ([120 150 230]+0)/383;c3 = ([120 150 230]+128)/383;patch([0 1 1 0],[0 0 1 1],c1);patch([0 1 1 1-e 1-e 0+e],[0 0 1 1-e 0+e 0+e],c2);patch([0 0 1 1-e 0+e 0+e],[0 1 1 1-e 1-e 0+e],c3);plot([0 1 1 0 0],[0 0 1 1 0]);disp('weights');
  "IW{2,1}(732,:)'" : Constant  Value=[0.214694094124904477638438038411550223827362060546875;-0.1489408644795472691502169482191675342619419097900390625;0.82711425787096926054431378361186943948268890380859375;-2.579469886217237384329337146482430398464202880859375;1.49451533315321594130864468752406537532806396484375;-0.827471181024518553925872765830717980861663818359375;0.36106840765111847257884392092819325625896453857421875;-0.9548669151003899013829823161358945071697235107421875]
      mask Display: e = 0.06;c1 = [120 150 230]/255;c2 = ([120 150 230]+0)/383;c3 = ([120 150 230]+128)/383;patch([0 1 1 0],[0 0 1 1],c1);patch([0 1 1 1-e 1-e 0+e],[0 0 1 1-e 0+e 0+e],c2);patch([0 0 1 1-e 0+e 0+e],[0 1 1 1-e 1-e 0+e],c3);plot([0 1 1 0 0],[0 0 1 1 0]);disp('weights');
  "IW{2,1}(733,:)'" : Constant  Value=[1.2920343926513766508179514858056791126728057861328125;0.219226266631392940897882226636284030973911285400390625;-0.049135609157929464874126068707482772879302501678466796875;-1.3053617696803903047708672602311708033084869384765625;1.25495448058603198404625800321809947490692138671875;1.1193965404560477505668814046657644212245941162109375;-1.5441741337855763305242362548597157001495361328125;1.5443263362718353537417215193272568285465240478515625]
      mask Display: e = 0.06;c1 = [120 150 230]/255;c2 = ([120 150 230]+0)/383;c3 = ([120 150 230]+128)/383;patch([0 1 1 0],[0 0 1 1],c1);patch([0 1 1 1-e 1-e 0+e],[0 0 1 1-e 0+e 0+e],c2);patch([0 0 1 1-e 0+e 0+e],[0 1 1 1-e 1-e 0+e],c3);plot([0 1 1 0 0],[0 0 1 1 0]);disp('weights');
  "IW{2,1}(734,:)'" : Constant  Value=[-1.06297138058298656915212632156908512115478515625;-1.10510609263221315501368735567666590213775634765625;1.28613637868959518328892954741604626178741455078125;1.3367963963464066790010065233218483626842498779296875;1.3643530864549460179802053971798159182071685791015625;0.2401204366879693685721264273524866439402103424072265625;-1.6156236758273128106822014160570688545703887939453125;0.823613369388225269318581922561861574649810791015625]
      mask Display: e = 0.06;c1 = [120 150 230]/255;c2 = ([120 150 230]+0)/383;c3 = ([120 150 230]+128)/383;patch([0 1 1 0],[0 0 1 1],c1);patch([0 1 1 1-e 1-e 0+e],[0 0 1 1-e 0+e 0+e],c2);patch([0 0 1 1-e 0+e 0+e],[0 1 1 1-e 1-e 0+e],c3);plot([0 1 1 0 0],[0 0 1 1 0]);disp('weights');
  "IW{2,1}(735,:)'" : Constant  Value=[-0.94734448852855834832809023282607086002826690673828125;0.61609105407661945985609008857863955199718475341796875;1.8716114179741436540638233054778538644313812255859375;-0.8275216647041203632539918544352985918521881103515625;0.94308987033098901076044739966164343059062957763671875;-0.4944808964041438326120214696857146918773651123046875;1.9648218982374852092931405422859825193881988525390625;-0.6062906335417945768995195976458489894866943359375]
      mask Display: e = 0.06;c1 = [120 150 230]/255;c2 = ([120 150 230]+0)/383;c3 = ([120 150 230]+128)/383;patch([0 1 1 0],[0 0 1 1],c1);patch([0 1 1 1-e 1-e 0+e],[0 0 1 1-e 0+e 0+e],c2);patch([0 0 1 1-e 0+e 0+e],[0 1 1 1-e 1-e 0+e],c3);plot([0 1 1 0 0],[0 0 1 1 0]);disp('weights');
  "IW{2,1}(736,:)'" : Constant  Value=[-1.806501016625265521042820182628929615020751953125;1.2680102059847848661178204565658234059810638427734375;-1.654026303287599919400463477359153330326080322265625;-1.3514743203272294724825997036532498896121978759765625;0.203225607537985630823840210723574273288249969482421875;-0.160258021772221981304795690448372624814510345458984375;-1.1354390701896919235736049813567660748958587646484375;0.475065903483182838673570813625701703131198883056640625]
      mask Display: e = 0.06;c1 = [120 150 230]/255;c2 = ([120 150 230]+0)/383;c3 = ([120 150 230]+128)/383;patch([0 1 1 0],[0 0 1 1],c1);patch([0 1 1 1-e 1-e 0+e],[0 0 1 1-e 0+e 0+e],c2);patch([0 0 1 1-e 0+e 0+e],[0 1 1 1-e 1-e 0+e],c3);plot([0 1 1 0 0],[0 0 1 1 0]);disp('weights');
  "IW{2,1}(737,:)'" : Constant  Value=[0.2271597656275458898544883368231239728629589080810546875;0.1829810474938735609384821145795285701751708984375;0.1872100206904807884189523292661760933697223663330078125;0.04949465009401242399089682066914974711835384368896484375;-1.9510876298485551050276853857212699949741363525390625;-1.24080333948038035174477045075036585330963134765625;2.286094029662951054859831856447272002696990966796875;0.7725908512515313741886302523198537528514862060546875]
      mask Display: e = 0.06;c1 = [120 150 230]/255;c2 = ([120 150 230]+0)/383;c3 = ([120 150 230]+128)/383;patch([0 1 1 0],[0 0 1 1],c1);patch([0 1 1 1-e 1-e 0+e],[0 0 1 1-e 0+e 0+e],c2);patch([0 0 1 1-e 0+e 0+e],[0 1 1 1-e 1-e 0+e],c3);plot([0 1 1 0 0],[0 0 1 1 0]);disp('weights');
  "IW{2,1}(738,:)'" : Constant  Value=[-0.90911900581571780666223503430956043303012847900390625;-1.385649697955340986510464063030667603015899658203125;1.565650646544526569670097160269506275653839111328125;1.086999841160615432045233319513499736785888671875;-1.5663842919342940707139177902718074619770050048828125;-0.776044598052585410385972863878123462200164794921875;0.87801399669547042226014355037477798759937286376953125;0.95311538142149465624441972977365367114543914794921875]
      mask Display: e = 0.06;c1 = [120 150 230]/255;c2 = ([120 150 230]+0)/383;c3 = ([120 150 230]+128)/383;patch([0 1 1 0],[0 0 1 1],c1);patch([0 1 1 1-e 1-e 0+e],[0 0 1 1-e 0+e 0+e],c2);patch([0 0 1 1-e 0+e 0+e],[0 1 1 1-e 1-e 0+e],c3);plot([0 1 1 0 0],[0 0 1 1 0]);disp('weights');
  "IW{2,1}(739,:)'" : Constant  Value=[0.56930180736533342322758244336000643670558929443359375;-1.4792716707112234519883031680365093052387237548828125;-1.2078586818639249766960119814029894769191741943359375;1.6346774730128290631370191476889885962009429931640625;1.0952427490968281720284949187771417200565338134765625;-0.52885676194682462725182858775951899588108062744140625;-1.657471010174025760619542779750190675258636474609375;0.339603888326835468003395135383470915257930755615234375]
      mask Display: e = 0.06;c1 = [120 150 230]/255;c2 = ([120 150 230]+0)/383;c3 = ([120 150 230]+128)/383;patch([0 1 1 0],[0 0 1 1],c1);patch([0 1 1 1-e 1-e 0+e],[0 0 1 1-e 0+e 0+e],c2);patch([0 0 1 1-e 0+e 0+e],[0 1 1 1-e 1-e 0+e],c3);plot([0 1 1 0 0],[0 0 1 1 0]);disp('weights');
  "IW{2,1}(74,:)'" : Constant  Value=[-1.5042593528692498328069859780953265726566314697265625;1.2638443812061515014733004136360250413417816162109375;1.2570179857374308429740494830184616148471832275390625;-1.47950414523176476677690516225993633270263671875;0.86437386242121949653238743849215097725391387939453125;-1.189576610856012184314067781087942421436309814453125;-0.37062537239830939395091036203666590154170989990234375;-1.122527608284979994124341828864999115467071533203125]
      mask Display: e = 0.06;c1 = [120 150 230]/255;c2 = ([120 150 230]+0)/383;c3 = ([120 150 230]+128)/383;patch([0 1 1 0],[0 0 1 1],c1);patch([0 1 1 1-e 1-e 0+e],[0 0 1 1-e 0+e 0+e],c2);patch([0 0 1 1-e 0+e 0+e],[0 1 1 1-e 1-e 0+e],c3);plot([0 1 1 0 0],[0 0 1 1 0]);disp('weights');
  "IW{2,1}(740,:)'" : Constant  Value=[-0.96165155849391792397540257297805510461330413818359375;1.89911483174009543262172883260063827037811279296875;0.1327552923598405432148439331285771913826465606689453125;1.1554295371111729107127530369325540959835052490234375;1.8674089223062619868898082131636328995227813720703125;-0.08243146470137786840925997466911212541162967681884765625;-0.93190472473765328942363339592702686786651611328125;-0.9684887534060404590263715363107621669769287109375]
      mask Display: e = 0.06;c1 = [120 150 230]/255;c2 = ([120 150 230]+0)/383;c3 = ([120 150 230]+128)/383;patch([0 1 1 0],[0 0 1 1],c1);patch([0 1 1 1-e 1-e 0+e],[0 0 1 1-e 0+e 0+e],c2);patch([0 0 1 1-e 0+e 0+e],[0 1 1 1-e 1-e 0+e],c3);plot([0 1 1 0 0],[0 0 1 1 0]);disp('weights');
  "IW{2,1}(741,:)'" : Constant  Value=[1.3605976303851807784894845099188387393951416015625;-0.42869430462441437956755407867603935301303863525390625;0.499775294136416137202871823319583199918270111083984375;0.235569645896044732591434467394719831645488739013671875;-0.47613465688641121165147751526092179119586944580078125;1.7071739142662278876372283775708638131618499755859375;1.681130669948843969763174754916690289974212646484375;-1.640029804090243459313569474034011363983154296875]
      mask Display: e = 0.06;c1 = [120 150 230]/255;c2 = ([120 150 230]+0)/383;c3 = ([120 150 230]+128)/383;patch([0 1 1 0],[0 0 1 1],c1);patch([0 1 1 1-e 1-e 0+e],[0 0 1 1-e 0+e 0+e],c2);patch([0 0 1 1-e 0+e 0+e],[0 1 1 1-e 1-e 0+e],c3);plot([0 1 1 0 0],[0 0 1 1 0]);disp('weights');
  "IW{2,1}(742,:)'" : Constant  Value=[-1.02136311104749211153830401599407196044921875;-0.59486917577850018101770501743885688483715057373046875;0.81963743308279812804784114632639102637767791748046875;1.782666221868260958416385619784705340862274169921875;-0.9151625619852106208185205105110071599483489990234375;-0.97500795001217166468876484941574744880199432373046875;-1.5806015350380351325298988740541972219944000244140625;-1.2150218779764438981061402955674566328525543212890625]
      mask Display: e = 0.06;c1 = [120 150 230]/255;c2 = ([120 150 230]+0)/383;c3 = ([120 150 230]+128)/383;patch([0 1 1 0],[0 0 1 1],c1);patch([0 1 1 1-e 1-e 0+e],[0 0 1 1-e 0+e 0+e],c2);patch([0 0 1 1-e 0+e 0+e],[0 1 1 1-e 1-e 0+e],c3);plot([0 1 1 0 0],[0 0 1 1 0]);disp('weights');
  "IW{2,1}(743,:)'" : Constant  Value=[1.681599557434028557878491483279503881931304931640625;-1.0675319852304101519990808810689486563205718994140625;-0.51551099987596582518989407617482356727123260498046875;0.004286627687641567270582232396236577187664806842803955078125;-1.4710187970360764087018878853996284306049346923828125;-1.270144983596825927207873974111862480640411376953125;-0.7502026211081844753181258056429214775562286376953125;1.521390580776149636932359499041922390460968017578125]
      mask Display: e = 0.06;c1 = [120 150 230]/255;c2 = ([120 150 230]+0)/383;c3 = ([120 150 230]+128)/383;patch([0 1 1 0],[0 0 1 1],c1);patch([0 1 1 1-e 1-e 0+e],[0 0 1 1-e 0+e 0+e],c2);patch([0 0 1 1-e 0+e 0+e],[0 1 1 1-e 1-e 0+e],c3);plot([0 1 1 0 0],[0 0 1 1 0]);disp('weights');
  "IW{2,1}(744,:)'" : Constant  Value=[0.1308287348547081674343672830218565650284290313720703125;-1.1331000290885244741190263084718026220798492431640625;0.64231531485877935150341500047943554818630218505859375;1.5320148752739821684798471324029378592967987060546875;-1.3085231717081582392125937985838390886783599853515625;-0.404262354232081511096197345977998338639736175537109375;0.08793811378879438922506750486718374304473400115966796875;-2.218410041487342443389252366614528000354766845703125]
      mask Display: e = 0.06;c1 = [120 150 230]/255;c2 = ([120 150 230]+0)/383;c3 = ([120 150 230]+128)/383;patch([0 1 1 0],[0 0 1 1],c1);patch([0 1 1 1-e 1-e 0+e],[0 0 1 1-e 0+e 0+e],c2);patch([0 0 1 1-e 0+e 0+e],[0 1 1 1-e 1-e 0+e],c3);plot([0 1 1 0 0],[0 0 1 1 0]);disp('weights');
  "IW{2,1}(745,:)'" : Constant  Value=[-1.9672107400736127402751662884838879108428955078125;-0.4798008457671425475155047024600207805633544921875;-0.031419120707542713688553703832440078258514404296875;0.897982434521970684926372996415011584758758544921875;-1.0159817487130471391765240696258842945098876953125;-1.374477095331492204621781638707034289836883544921875;-1.7530507125619030350804905538097955286502838134765625;0.361886587511485002810474043144495226442813873291015625]
      mask Display: e = 0.06;c1 = [120 150 230]/255;c2 = ([120 150 230]+0)/383;c3 = ([120 150 230]+128)/383;patch([0 1 1 0],[0 0 1 1],c1);patch([0 1 1 1-e 1-e 0+e],[0 0 1 1-e 0+e 0+e],c2);patch([0 0 1 1-e 0+e 0+e],[0 1 1 1-e 1-e 0+e],c3);plot([0 1 1 0 0],[0 0 1 1 0]);disp('weights');
  "IW{2,1}(746,:)'" : Constant  Value=[-1.5997089570347367004643501786631532013416290283203125;0.8490685444049075325523290302953682839870452880859375;-0.17063437232296585488455775703187100589275360107421875;1.4516170450808802971920385971316136419773101806640625;-2.099536259164961560230722170672379434108734130859375;0.03557102441952599003460733229076140560209751129150390625;-0.6909064645609730437314510709256865084171295166015625;-0.8338098182474948938391889896593056619167327880859375]
      mask Display: e = 0.06;c1 = [120 150 230]/255;c2 = ([120 150 230]+0)/383;c3 = ([120 150 230]+128)/383;patch([0 1 1 0],[0 0 1 1],c1);patch([0 1 1 1-e 1-e 0+e],[0 0 1 1-e 0+e 0+e],c2);patch([0 0 1 1-e 0+e 0+e],[0 1 1 1-e 1-e 0+e],c3);plot([0 1 1 0 0],[0 0 1 1 0]);disp('weights');
  "IW{2,1}(747,:)'" : Constant  Value=[1.930248741364115172558513222611509263515472412109375;-0.54004379796680834768807244472554884850978851318359375;0.209517274755824878251786458349670283496379852294921875;1.276260843325605964793112434563226997852325439453125;0.99591537568212007425216825140523724257946014404296875;-0.48846647394042719270146335475146770477294921875;-0.9097959195975608981399318508920259773731231689453125;1.825238102829378927793868570006452500820159912109375]
      mask Display: e = 0.06;c1 = [120 150 230]/255;c2 = ([120 150 230]+0)/383;c3 = ([120 150 230]+128)/383;patch([0 1 1 0],[0 0 1 1],c1);patch([0 1 1 1-e 1-e 0+e],[0 0 1 1-e 0+e 0+e],c2);patch([0 0 1 1-e 0+e 0+e],[0 1 1 1-e 1-e 0+e],c3);plot([0 1 1 0 0],[0 0 1 1 0]);disp('weights');
  "IW{2,1}(748,:)'" : Constant  Value=[-1.007041497159892884383225464262068271636962890625;1.408742826053984931178320039180107414722442626953125;-0.3090213716654226505653468848322518169879913330078125;-1.2780961209198782313478659489192068576812744140625;-0.8874937526154640377029636510997079312801361083984375;1.032812801842294181398074215394444763660430908203125;1.6651125367807420030175080682965926826000213623046875;-1.44177488277090848356465357937850058078765869140625]
      mask Display: e = 0.06;c1 = [120 150 230]/255;c2 = ([120 150 230]+0)/383;c3 = ([120 150 230]+128)/383;patch([0 1 1 0],[0 0 1 1],c1);patch([0 1 1 1-e 1-e 0+e],[0 0 1 1-e 0+e 0+e],c2);patch([0 0 1 1-e 0+e 0+e],[0 1 1 1-e 1-e 0+e],c3);plot([0 1 1 0 0],[0 0 1 1 0]);disp('weights');
  "IW{2,1}(749,:)'" : Constant  Value=[0.60608405180481550456050854336353950202465057373046875;-1.879352996953799870283319251029752194881439208984375;-0.2240625096960423279224272619103430770337581634521484375;-1.726131659323292044661002364591695368289947509765625;-0.13201797357477140781867319674347527325153350830078125;1.30234048105892963320684430073015391826629638671875;1.6013917512039113066890649861306883394718170166015625;0.038676776170386950592927632897044532001018524169921875]
      mask Display: e = 0.06;c1 = [120 150 230]/255;c2 = ([120 150 230]+0)/383;c3 = ([120 150 230]+128)/383;patch([0 1 1 0],[0 0 1 1],c1);patch([0 1 1 1-e 1-e 0+e],[0 0 1 1-e 0+e 0+e],c2);patch([0 0 1 1-e 0+e 0+e],[0 1 1 1-e 1-e 0+e],c3);plot([0 1 1 0 0],[0 0 1 1 0]);disp('weights');
  "IW{2,1}(75,:)'" : Constant  Value=[1.4533874673690945211745884080301038920879364013671875;1.3876264208173108016808328102342784404754638671875;1.55080341271489086096835308126173913478851318359375;1.4141742333968896350171462472644634544849395751953125;-0.2850690801581385880325569814885966479778289794921875;-1.2259906141338152707476183422841131687164306640625;-1.022087514937825236671642414876259863376617431640625;0.36796909427792423574743452263646759092807769775390625]
      mask Display: e = 0.06;c1 = [120 150 230]/255;c2 = ([120 150 230]+0)/383;c3 = ([120 150 230]+128)/383;patch([0 1 1 0],[0 0 1 1],c1);patch([0 1 1 1-e 1-e 0+e],[0 0 1 1-e 0+e 0+e],c2);patch([0 0 1 1-e 0+e 0+e],[0 1 1 1-e 1-e 0+e],c3);plot([0 1 1 0 0],[0 0 1 1 0]);disp('weights');
  "IW{2,1}(750,:)'" : Constant  Value=[-0.48031015178603564397263880891841836273670196533203125;0.448687531881742984740668589438428170979022979736328125;-0.424631851982952113200298072115401737391948699951171875;2.195795741185153193697487949975766241550445556640625;0.763353543224744246487034615711309015750885009765625;0.51248338422156347604641268844716250896453857421875;1.4892615942150178032221674584434367716312408447265625;-1.572065855518613997077181920758448541164398193359375]
      mask Display: e = 0.06;c1 = [120 150 230]/255;c2 = ([120 150 230]+0)/383;c3 = ([120 150 230]+128)/383;patch([0 1 1 0],[0 0 1 1],c1);patch([0 1 1 1-e 1-e 0+e],[0 0 1 1-e 0+e 0+e],c2);patch([0 0 1 1-e 0+e 0+e],[0 1 1 1-e 1-e 0+e],c3);plot([0 1 1 0 0],[0 0 1 1 0]);disp('weights');
  "IW{2,1}(751,:)'" : Constant  Value=[0.955642930270370616341324421227909624576568603515625;0.12291919887550505074980122799388482235372066497802734375;1.5628547983063771908973649260587990283966064453125;1.4010941973349277933635903536924161016941070556640625;0.282986026122756417766623826537397690117359161376953125;-0.78840431277062361647978150358540005981922149658203125;-1.337039758306258985243175629875622689723968505859375;1.786447489931278997943309150286950170993804931640625]
      mask Display: e = 0.06;c1 = [120 150 230]/255;c2 = ([120 150 230]+0)/383;c3 = ([120 150 230]+128)/383;patch([0 1 1 0],[0 0 1 1],c1);patch([0 1 1 1-e 1-e 0+e],[0 0 1 1-e 0+e 0+e],c2);patch([0 0 1 1-e 0+e 0+e],[0 1 1 1-e 1-e 0+e],c3);plot([0 1 1 0 0],[0 0 1 1 0]);disp('weights');
  "IW{2,1}(752,:)'" : Constant  Value=[0.054181072387849450733288136916598887182772159576416015625;-1.50784811412479857750668088556267321109771728515625;0.58109506848123959610319388957577757537364959716796875;1.794447807459906840676922001875936985015869140625;-0.07763337124022375024257058839793899096548557281494140625;0.0704516293304175145184586881441646255552768707275390625;-0.8993320165465317206354711743188090622425079345703125;2.109828248244550508161410107277333736419677734375]
      mask Display: e = 0.06;c1 = [120 150 230]/255;c2 = ([120 150 230]+0)/383;c3 = ([120 150 230]+128)/383;patch([0 1 1 0],[0 0 1 1],c1);patch([0 1 1 1-e 1-e 0+e],[0 0 1 1-e 0+e 0+e],c2);patch([0 0 1 1-e 0+e 0+e],[0 1 1 1-e 1-e 0+e],c3);plot([0 1 1 0 0],[0 0 1 1 0]);disp('weights');
